simulink model "untitled1"  (R2019b)
(part 13 of 13)

      mask Display: e = 0.06;c1 = [120 150 230]/255;c2 = ([120 150 230]+0)/383;c3 = ([120 150 230]+128)/383;patch([0 1 1 0],[0 0 1 1],c1);patch([0 1 1 1-e 1-e 0+e],[0 0 1 1-e 0+e 0+e],c2);patch([0 0 1 1-e 0+e 0+e],[0 1 1 1-e 1-e 0+e],c3);plot([0 1 1 0 0],[0 0 1 1 0]);disp('weights');
  "IW{2,1}(965,:)'" : Constant  Value=[-0.7144394409110896848602578756981529295444488525390625;0.3471428091304182839138547933544032275676727294921875;0.7770557749069857411683415193692781031131744384765625;0.884710969750206910333645282662473618984222412109375;-0.848870413859076133888947879313491284847259521484375;-0.5348404016948873351822157928836531937122344970703125;0.9006006133464066198968112075817771255970001220703125;0.6799960425277957742906664861948229372501373291015625;-0.4140176799412766950325703874113969504833221435546875;0.9711691691262831493958174178260378539562225341796875]
      mask Display: e = 0.06;c1 = [120 150 230]/255;c2 = ([120 150 230]+0)/383;c3 = ([120 150 230]+128)/383;patch([0 1 1 0],[0 0 1 1],c1);patch([0 1 1 1-e 1-e 0+e],[0 0 1 1-e 0+e 0+e],c2);patch([0 0 1 1-e 0+e 0+e],[0 1 1 1-e 1-e 0+e],c3);plot([0 1 1 0 0],[0 0 1 1 0]);disp('weights');
  "IW{2,1}(966,:)'" : Constant  Value=[-0.01557806455447430238336892216466367244720458984375;-0.5368941087142620194327946592238731682300567626953125;-0.618426386315975573637615525512956082820892333984375;-0.387222706560339080539279166259802877902984619140625;0.6692859941373978660550392305594868957996368408203125;-0.7869100555616228565014580453862436115741729736328125;-0.4994862083211952796801824661088176071643829345703125;-0.5272965717421425058120121320826001465320587158203125;-0.4900147760632862503626938632805831730365753173828125;-0.9665330389173429903593159906449727714061737060546875]
      mask Display: e = 0.06;c1 = [120 150 230]/255;c2 = ([120 150 230]+0)/383;c3 = ([120 150 230]+128)/383;patch([0 1 1 0],[0 0 1 1],c1);patch([0 1 1 1-e 1-e 0+e],[0 0 1 1-e 0+e 0+e],c2);patch([0 0 1 1-e 0+e 0+e],[0 1 1 1-e 1-e 0+e],c3);plot([0 1 1 0 0],[0 0 1 1 0]);disp('weights');
  "IW{2,1}(967,:)'" : Constant  Value=[-0.984051897323352076085711814812384545803070068359375;-0.7181505786073738573094260573270730674266815185546875;0.6028705818402577687464827249641530215740203857421875;-0.3125907138719998812348421779461205005645751953125;-0.646850905156462818723639429663307964801788330078125;-0.1469398150759413379518036890658549964427947998046875;-0.4738723005891622985785716082318685948848724365234375;0.172262093721131659407319602905772626399993896484375;0.1993207325021995046654410543851554393768310546875;-0.698448571765098780161906688590534031391143798828125]
      mask Display: e = 0.06;c1 = [120 150 230]/255;c2 = ([120 150 230]+0)/383;c3 = ([120 150 230]+128)/383;patch([0 1 1 0],[0 0 1 1],c1);patch([0 1 1 1-e 1-e 0+e],[0 0 1 1-e 0+e 0+e],c2);patch([0 0 1 1-e 0+e 0+e],[0 1 1 1-e 1-e 0+e],c3);plot([0 1 1 0 0],[0 0 1 1 0]);disp('weights');
  "IW{2,1}(968,:)'" : Constant  Value=[-0.04533156631802004454812049516476690769195556640625;0.70667647898809438089529066928662359714508056640625;0.1328876134866188163385913867386989295482635498046875;-0.17361026655103017901637940667569637298583984375;-0.040194056538962019686778148752637207508087158203125;-0.256956070446161977116616981220431625843048095703125;0.5707768518799058998780537876882590353488922119140625;0.51234341589951792883539383183233439922332763671875;0.2440885450435192893792191171087324619293212890625;-0.3020562993950519636854323834995739161968231201171875]
      mask Display: e = 0.06;c1 = [120 150 230]/255;c2 = ([120 150 230]+0)/383;c3 = ([120 150 230]+128)/383;patch([0 1 1 0],[0 0 1 1],c1);patch([0 1 1 1-e 1-e 0+e],[0 0 1 1-e 0+e 0+e],c2);patch([0 0 1 1-e 0+e 0+e],[0 1 1 1-e 1-e 0+e],c3);plot([0 1 1 0 0],[0 0 1 1 0]);disp('weights');
  "IW{2,1}(969,:)'" : Constant  Value=[-0.11648547445748480555494097643531858921051025390625;0.4586267717677987576507803169079124927520751953125;-0.511564703530516862173271874780766665935516357421875;-0.1978762319989491036409390289918519556522369384765625;0.324395333392201390410036765388213098049163818359375;0.10679205805803793083441632916219532489776611328125;0.58851580401107117523906708811409771442413330078125;0.24338547710045244087950777611695230007171630859375;0.621085435282426434611124932416714727878570556640625;-0.531323053611133300222491016029380261898040771484375]
      mask Display: e = 0.06;c1 = [120 150 230]/255;c2 = ([120 150 230]+0)/383;c3 = ([120 150 230]+128)/383;patch([0 1 1 0],[0 0 1 1],c1);patch([0 1 1 1-e 1-e 0+e],[0 0 1 1-e 0+e 0+e],c2);patch([0 0 1 1-e 0+e 0+e],[0 1 1 1-e 1-e 0+e],c3);plot([0 1 1 0 0],[0 0 1 1 0]);disp('weights');
  "IW{2,1}(97,:)'" : Constant  Value=[0.5164505764297786516436872261692769825458526611328125;0.98169912664928471457415071199648082256317138671875;-0.0315123656142617392106330953538417816162109375;0.191559320614675510086044596391730010509490966796875;0.996933890817953027863040915690362453460693359375;0.9568910074119532094272244648891501128673553466796875;-0.156110393169701211490973946638405323028564453125;0.5571506750401284957519010276882909238338470458984375;-0.4503567660380503046013700441108085215091705322265625;0.3282242045748076098021783764124847948551177978515625]
      mask Display: e = 0.06;c1 = [120 150 230]/255;c2 = ([120 150 230]+0)/383;c3 = ([120 150 230]+128)/383;patch([0 1 1 0],[0 0 1 1],c1);patch([0 1 1 1-e 1-e 0+e],[0 0 1 1-e 0+e 0+e],c2);patch([0 0 1 1-e 0+e 0+e],[0 1 1 1-e 1-e 0+e],c3);plot([0 1 1 0 0],[0 0 1 1 0]);disp('weights');
  "IW{2,1}(970,:)'" : Constant  Value=[0.66557065240704016417794264270924031734466552734375;-0.342585064829493912696989355026744306087493896484375;-0.330671300947106061585145653225481510162353515625;0.763105148353479645351171711809001863002777099609375;-0.847724061807384909883467116742394864559173583984375;-0.7336611657769716021704198283259756863117218017578125;-0.8233078430220610588463614476495422422885894775390625;0.944306077394880372111174438032321631908416748046875;-0.8467439093702473495994809127296321094036102294921875;0.365460195039065904865083211916498839855194091796875]
      mask Display: e = 0.06;c1 = [120 150 230]/255;c2 = ([120 150 230]+0)/383;c3 = ([120 150 230]+128)/383;patch([0 1 1 0],[0 0 1 1],c1);patch([0 1 1 1-e 1-e 0+e],[0 0 1 1-e 0+e 0+e],c2);patch([0 0 1 1-e 0+e 0+e],[0 1 1 1-e 1-e 0+e],c3);plot([0 1 1 0 0],[0 0 1 1 0]);disp('weights');
  "IW{2,1}(971,:)'" : Constant  Value=[0.09986387496097304250497472821734845638275146484375;-0.83951506989385205059761574375443160533905029296875;0.3955738003209976483276477665640413761138916015625;-0.339458412070430259888098589726723730564117431640625;-0.3938174570716068689790745338541455566883087158203125;-0.5670824324329546417544634095975197851657867431640625;0.1650021316949297212062219841754995286464691162109375;-0.562756802057183147525165622937493026256561279296875;-0.794803053725064767576213853317312896251678466796875;-0.6683564360248277491649560033692978322505950927734375]
      mask Display: e = 0.06;c1 = [120 150 230]/255;c2 = ([120 150 230]+0)/383;c3 = ([120 150 230]+128)/383;patch([0 1 1 0],[0 0 1 1],c1);patch([0 1 1 1-e 1-e 0+e],[0 0 1 1-e 0+e 0+e],c2);patch([0 0 1 1-e 0+e 0+e],[0 1 1 1-e 1-e 0+e],c3);plot([0 1 1 0 0],[0 0 1 1 0]);disp('weights');
  "IW{2,1}(972,:)'" : Constant  Value=[0.268960675494376300065368923242203891277313232421875;0.4899821727860824704947617647121660411357879638671875;0.6479216729186567658160811333800666034221649169921875;0.0558113266099151683619083996745757758617401123046875;-0.6532374748577816081507307899300940334796905517578125;0.8237949914928128780644556172774173319339752197265625;-0.2383918818598125266561282842303626239299774169921875;0.9738616798149990483324245360563509166240692138671875;0.871706348437010003493696785881184041500091552734375;-0.5074443580581782242688859696500003337860107421875]
      mask Display: e = 0.06;c1 = [120 150 230]/255;c2 = ([120 150 230]+0)/383;c3 = ([120 150 230]+128)/383;patch([0 1 1 0],[0 0 1 1],c1);patch([0 1 1 1-e 1-e 0+e],[0 0 1 1-e 0+e 0+e],c2);patch([0 0 1 1-e 0+e 0+e],[0 1 1 1-e 1-e 0+e],c3);plot([0 1 1 0 0],[0 0 1 1 0]);disp('weights');
  "IW{2,1}(973,:)'" : Constant  Value=[0.675627511982876516327678473317064344882965087890625;0.4241577164580718761754951628972776234149932861328125;-0.448557670053332913084886968135833740234375;-0.7164721751960041462581330051762051880359649658203125;-0.2684544674326294622090927077806554734706878662109375;0.54120202347532231357263299287296831607818603515625;0.5901741429993838661260951994336210191249847412109375;-0.2376909062983745268837765252101235091686248779296875;0.285221199923347601412615404115058481693267822265625;0.2521625711384434254114239593036472797393798828125]
      mask Display: e = 0.06;c1 = [120 150 230]/255;c2 = ([120 150 230]+0)/383;c3 = ([120 150 230]+128)/383;patch([0 1 1 0],[0 0 1 1],c1);patch([0 1 1 1-e 1-e 0+e],[0 0 1 1-e 0+e 0+e],c2);patch([0 0 1 1-e 0+e 0+e],[0 1 1 1-e 1-e 0+e],c3);plot([0 1 1 0 0],[0 0 1 1 0]);disp('weights');
  "IW{2,1}(974,:)'" : Constant  Value=[-0.5093344195065017121493156082578934729099273681640625;-0.122100702365118163328361333697102963924407958984375;-0.06613544440721597084120730869472026824951171875;0.85418845517627328689513888093642890453338623046875;0.1864830168329245640990166066330857574939727783203125;-0.1153004956934562397208310358109883964061737060546875;0.7030618126919361277060716020059771835803985595703125;0.9119188834696230205878464403213001787662506103515625;0.0358341940688620130828212495543994009494781494140625;0.2699457411017520680474035543738864362239837646484375]
      mask Display: e = 0.06;c1 = [120 150 230]/255;c2 = ([120 150 230]+0)/383;c3 = ([120 150 230]+128)/383;patch([0 1 1 0],[0 0 1 1],c1);patch([0 1 1 1-e 1-e 0+e],[0 0 1 1-e 0+e 0+e],c2);patch([0 0 1 1-e 0+e 0+e],[0 1 1 1-e 1-e 0+e],c3);plot([0 1 1 0 0],[0 0 1 1 0]);disp('weights');
  "IW{2,1}(975,:)'" : Constant  Value=[-0.44832821462690386482563553727231919765472412109375;-0.581481593458495371606886692461557686328887939453125;-0.8669823002726253502459030642057769000530242919921875;0.4658169283180739750349630412529222667217254638671875;0.9658499535101270350168078948627226054668426513671875;0.554359087851052922957251212210394442081451416015625;0.3636363138170199960086392820812761783599853515625;0.047593285412130370559680159203708171844482421875;0.468161357721236459639158056234009563922882080078125;-0.618507986207100568520900196745060384273529052734375]
      mask Display: e = 0.06;c1 = [120 150 230]/255;c2 = ([120 150 230]+0)/383;c3 = ([120 150 230]+128)/383;patch([0 1 1 0],[0 0 1 1],c1);patch([0 1 1 1-e 1-e 0+e],[0 0 1 1-e 0+e 0+e],c2);patch([0 0 1 1-e 0+e 0+e],[0 1 1 1-e 1-e 0+e],c3);plot([0 1 1 0 0],[0 0 1 1 0]);disp('weights');
  "IW{2,1}(976,:)'" : Constant  Value=[0.63512671701889278352837209240533411502838134765625;0.76995771079419395022114258608780801296234130859375;-0.3323635258169665984695484439725987613201141357421875;0.7269204450465860389840599964372813701629638671875;-0.4794860357969399355937412110506556928157806396484375;0.721878388283787586487960652448236942291259765625;0.5611042141713820097237430672976188361644744873046875;0.5470365148935558696763337138690985739231109619140625;0.524079115559971331350652690161950886249542236328125;0.5223507529721056474869556041085161268711090087890625]
      mask Display: e = 0.06;c1 = [120 150 230]/255;c2 = ([120 150 230]+0)/383;c3 = ([120 150 230]+128)/383;patch([0 1 1 0],[0 0 1 1],c1);patch([0 1 1 1-e 1-e 0+e],[0 0 1 1-e 0+e 0+e],c2);patch([0 0 1 1-e 0+e 0+e],[0 1 1 1-e 1-e 0+e],c3);plot([0 1 1 0 0],[0 0 1 1 0]);disp('weights');
  "IW{2,1}(977,:)'" : Constant  Value=[-0.661425562563644486857583615346811711788177490234375;0.881450618622593662365716227213852107524871826171875;0.5362793846547531106949691093177534639835357666015625;0.9636728247019397119998984635458327829837799072265625;-0.6788919886295976535706131471670232713222503662109375;-0.2454345244011097992853365212795324623584747314453125;-0.2134483663315069890131780994124710559844970703125;-0.507588810722410244125057943165302276611328125;-0.0191293381497643633082361702690832316875457763671875;0.1988419730259847195696920607588253915309906005859375]
      mask Display: e = 0.06;c1 = [120 150 230]/255;c2 = ([120 150 230]+0)/383;c3 = ([120 150 230]+128)/383;patch([0 1 1 0],[0 0 1 1],c1);patch([0 1 1 1-e 1-e 0+e],[0 0 1 1-e 0+e 0+e],c2);patch([0 0 1 1-e 0+e 0+e],[0 1 1 1-e 1-e 0+e],c3);plot([0 1 1 0 0],[0 0 1 1 0]);disp('weights');
  "IW{2,1}(978,:)'" : Constant  Value=[0.9397617197588667981023036190890707075595855712890625;-0.5050778654996699312818009275360964238643646240234375;-0.2310095659395277056802342485752888023853302001953125;-0.72151071109553921445467494777403771877288818359375;0.2458828822041303485690377783612348139286041259765625;-0.6318146365362140581822814056067727506160736083984375;0.493954060451254672869936257484368979930877685546875;-0.039417507091375370009700418449938297271728515625;-0.9730967142666300251363509232760407030582427978515625;-0.8911115925057833120348504962748847901821136474609375]
      mask Display: e = 0.06;c1 = [120 150 230]/255;c2 = ([120 150 230]+0)/383;c3 = ([120 150 230]+128)/383;patch([0 1 1 0],[0 0 1 1],c1);patch([0 1 1 1-e 1-e 0+e],[0 0 1 1-e 0+e 0+e],c2);patch([0 0 1 1-e 0+e 0+e],[0 1 1 1-e 1-e 0+e],c3);plot([0 1 1 0 0],[0 0 1 1 0]);disp('weights');
  "IW{2,1}(979,:)'" : Constant  Value=[-0.4741075419004106006326537681161426007747650146484375;0.205108870171887058830861860769800841808319091796875;0.29256486552897253972105318098329007625579833984375;0.7587563553566012419793196386308409273624420166015625;-0.375454775245055660803927821689285337924957275390625;0.231516223087936179325652119587175548076629638671875;0.070654245879933075258350072544999420642852783203125;0.83413919498149358133787245606072247028350830078125;0.6313603211407159410128997478750534355640411376953125;-0.85603804792848148252915052580647170543670654296875]
      mask Display: e = 0.06;c1 = [120 150 230]/255;c2 = ([120 150 230]+0)/383;c3 = ([120 150 230]+128)/383;patch([0 1 1 0],[0 0 1 1],c1);patch([0 1 1 1-e 1-e 0+e],[0 0 1 1-e 0+e 0+e],c2);patch([0 0 1 1-e 0+e 0+e],[0 1 1 1-e 1-e 0+e],c3);plot([0 1 1 0 0],[0 0 1 1 0]);disp('weights');
  "IW{2,1}(98,:)'" : Constant  Value=[-0.7749528854198344252068864079774357378482818603515625;-0.7248848268697927199610830939491279423236846923828125;-0.9015271498971679786649247034802101552486419677734375;0.3448050374539517459737680837861262261867523193359375;0.86952403079192475132686013239435851573944091796875;0.767582231090413902308000615448690950870513916015625;-0.64782980375393339755873967078514397144317626953125;0.517582748277408466464066805201582610607147216796875;0.9891107209328253713209733177791349589824676513671875;0.391932819643511454188455900293774902820587158203125]
      mask Display: e = 0.06;c1 = [120 150 230]/255;c2 = ([120 150 230]+0)/383;c3 = ([120 150 230]+128)/383;patch([0 1 1 0],[0 0 1 1],c1);patch([0 1 1 1-e 1-e 0+e],[0 0 1 1-e 0+e 0+e],c2);patch([0 0 1 1-e 0+e 0+e],[0 1 1 1-e 1-e 0+e],c3);plot([0 1 1 0 0],[0 0 1 1 0]);disp('weights');
  "IW{2,1}(980,:)'" : Constant  Value=[-0.79147398202981111836606942233629524707794189453125;0.2718975678685253694055745654623024165630340576171875;-0.4094504931238824863015679511590860784053802490234375;0.81854986253682682217913679778575897216796875;0.605274059499623096058940063812769949436187744140625;0.63404117958328409798696156940422952175140380859375;0.6294911340532147736581691788160242140293121337890625;-0.1480106713086433156689736279076896607875823974609375;0.93064947410425968854497114080004394054412841796875;0.93956211150475343885091206175275146961212158203125]
      mask Display: e = 0.06;c1 = [120 150 230]/255;c2 = ([120 150 230]+0)/383;c3 = ([120 150 230]+128)/383;patch([0 1 1 0],[0 0 1 1],c1);patch([0 1 1 1-e 1-e 0+e],[0 0 1 1-e 0+e 0+e],c2);patch([0 0 1 1-e 0+e 0+e],[0 1 1 1-e 1-e 0+e],c3);plot([0 1 1 0 0],[0 0 1 1 0]);disp('weights');
  "IW{2,1}(981,:)'" : Constant  Value=[-0.0852692222631059593140889774076640605926513671875;-0.899091542873903026844573105336166918277740478515625;-0.1471286623457948028459441047743894159793853759765625;-0.4211931943745510498189332793117500841617584228515625;0.36330329234651781433740325155667960643768310546875;-0.139104176957447922546862173476256430149078369140625;-0.7284662842966298512692446820437908172607421875;0.873058432394929528896909687318839132785797119140625;-0.605449246597180579243513420806266367435455322265625;-0.3582669903376476394640803846414200961589813232421875]
      mask Display: e = 0.06;c1 = [120 150 230]/255;c2 = ([120 150 230]+0)/383;c3 = ([120 150 230]+128)/383;patch([0 1 1 0],[0 0 1 1],c1);patch([0 1 1 1-e 1-e 0+e],[0 0 1 1-e 0+e 0+e],c2);patch([0 0 1 1-e 0+e 0+e],[0 1 1 1-e 1-e 0+e],c3);plot([0 1 1 0 0],[0 0 1 1 0]);disp('weights');
  "IW{2,1}(982,:)'" : Constant  Value=[-0.4342255528810079479029582216753624379634857177734375;0.172996624453667369181175672565586864948272705078125;0.2102942438550774451044844681746326386928558349609375;0.125405454503676683231105926097370684146881103515625;-0.9632340007484112565094847013824619352817535400390625;0.01979000329602786933946845238097012042999267578125;0.718517973057300363137755994102917611598968505859375;-0.358865564478632936840085676521994173526763916015625;0.3435920013824065311069944073096849024295806884765625;0.17049996845140835688425795524381101131439208984375]
      mask Display: e = 0.06;c1 = [120 150 230]/255;c2 = ([120 150 230]+0)/383;c3 = ([120 150 230]+128)/383;patch([0 1 1 0],[0 0 1 1],c1);patch([0 1 1 1-e 1-e 0+e],[0 0 1 1-e 0+e 0+e],c2);patch([0 0 1 1-e 0+e 0+e],[0 1 1 1-e 1-e 0+e],c3);plot([0 1 1 0 0],[0 0 1 1 0]);disp('weights');
  "IW{2,1}(983,:)'" : Constant  Value=[-0.1677270431949711149144377486663870513439178466796875;0.181662621682935565559091628529131412506103515625;0.851057986800337840094243802013806998729705810546875;-0.072748429997369523647421374334953725337982177734375;0.7882143648824444515099685304448939859867095947265625;0.4502981756526995837930371635593473911285400390625;0.1336104762519625399619371819426305592060089111328125;-0.9894179168451724404320657413336448371410369873046875;-0.60904986299242214187188437790609896183013916015625;0.555950035385905483309443297912366688251495361328125]
      mask Display: e = 0.06;c1 = [120 150 230]/255;c2 = ([120 150 230]+0)/383;c3 = ([120 150 230]+128)/383;patch([0 1 1 0],[0 0 1 1],c1);patch([0 1 1 1-e 1-e 0+e],[0 0 1 1-e 0+e 0+e],c2);patch([0 0 1 1-e 0+e 0+e],[0 1 1 1-e 1-e 0+e],c3);plot([0 1 1 0 0],[0 0 1 1 0]);disp('weights');
  "IW{2,1}(984,:)'" : Constant  Value=[-0.9698249573309529747433543889201246201992034912109375;-0.234376616891645017659584482316859066486358642578125;0.9737840786331359854699485367746092379093170166015625;0.8760765465004822782901783284614793956279754638671875;-0.024687881459021010499554904527030885219573974609375;-0.7129955988575460423817276023328304290771484375;-0.834665311211235660948659642599523067474365234375;0.838502337609266401585728090140037238597869873046875;0.8558601766537587973715517364325933158397674560546875;0.6368968800970955523865768554969690740108489990234375]
      mask Display: e = 0.06;c1 = [120 150 230]/255;c2 = ([120 150 230]+0)/383;c3 = ([120 150 230]+128)/383;patch([0 1 1 0],[0 0 1 1],c1);patch([0 1 1 1-e 1-e 0+e],[0 0 1 1-e 0+e 0+e],c2);patch([0 0 1 1-e 0+e 0+e],[0 1 1 1-e 1-e 0+e],c3);plot([0 1 1 0 0],[0 0 1 1 0]);disp('weights');
  "IW{2,1}(985,:)'" : Constant  Value=[-0.0091677671380521186250689424923621118068695068359375;0.800228653495768327275072806514799594879150390625;0.5410823945520999433966835567844100296497344970703125;-0.9494611157890806563131036455160938203334808349609375;-0.659980658289798238769208182930015027523040771484375;-0.00114901150523305517481276183389127254486083984375;-0.0136490491228522525801736264838837087154388427734375;-0.319972954472963255767581358668394386768341064453125;0.83703066722275121236407358082942664623260498046875;-0.444610457951165383150282650603912770748138427734375]
      mask Display: e = 0.06;c1 = [120 150 230]/255;c2 = ([120 150 230]+0)/383;c3 = ([120 150 230]+128)/383;patch([0 1 1 0],[0 0 1 1],c1);patch([0 1 1 1-e 1-e 0+e],[0 0 1 1-e 0+e 0+e],c2);patch([0 0 1 1-e 0+e 0+e],[0 1 1 1-e 1-e 0+e],c3);plot([0 1 1 0 0],[0 0 1 1 0]);disp('weights');
  "IW{2,1}(986,:)'" : Constant  Value=[0.8297443864155129578108471832820214331150054931640625;0.363935670188301418903620287892408668994903564453125;0.100383258658132579199673273251391947269439697265625;0.68812431176497401708047618740238249301910400390625;0.39841482140100747955102633568458259105682373046875;-0.5389940279242357856759326750761829316616058349609375;0.942748456213683194704344714409671723842620849609375;0.9881289869271363546232578300987370312213897705078125;-0.40606747251954455890654571703635156154632568359375;0.4138975726274001232241062098182737827301025390625]
      mask Display: e = 0.06;c1 = [120 150 230]/255;c2 = ([120 150 230]+0)/383;c3 = ([120 150 230]+128)/383;patch([0 1 1 0],[0 0 1 1],c1);patch([0 1 1 1-e 1-e 0+e],[0 0 1 1-e 0+e 0+e],c2);patch([0 0 1 1-e 0+e 0+e],[0 1 1 1-e 1-e 0+e],c3);plot([0 1 1 0 0],[0 0 1 1 0]);disp('weights');
  "IW{2,1}(987,:)'" : Constant  Value=[-0.99506550776042868022841503261588513851165771484375;0.68389640586497879581884262734092772006988525390625;-0.2268259999791315539852121219155378639698028564453125;-0.957738642747987256598207750357687473297119140625;0.26389345282455511920716162421740591526031494140625;-0.6102323831253475550084885981050319969654083251953125;-0.927066660789935159669994391151703894138336181640625;-0.549182384059821782074095608550123870372772216796875;0.0328332951849941157007606307161040604114532470703125;0.095697283614887940217386130825616419315338134765625]
      mask Display: e = 0.06;c1 = [120 150 230]/255;c2 = ([120 150 230]+0)/383;c3 = ([120 150 230]+128)/383;patch([0 1 1 0],[0 0 1 1],c1);patch([0 1 1 1-e 1-e 0+e],[0 0 1 1-e 0+e 0+e],c2);patch([0 0 1 1-e 0+e 0+e],[0 1 1 1-e 1-e 0+e],c3);plot([0 1 1 0 0],[0 0 1 1 0]);disp('weights');
  "IW{2,1}(988,:)'" : Constant  Value=[0.69592152169732468536267333547584712505340576171875;0.741406290005517387697864251094870269298553466796875;-0.8585444882144399603163265055627562105655670166015625;0.00846499148783852461974674952216446399688720703125;0.7336265843222864457828791273641400039196014404296875;-0.14664201888037897703043199726380407810211181640625;0.679580078540876542092519230209290981292724609375;-0.4031972201373006381430741384974680840969085693359375;-0.7367485188008242591450880354386754333972930908203125;-0.6177617192172204507727428790531121194362640380859375]
      mask Display: e = 0.06;c1 = [120 150 230]/255;c2 = ([120 150 230]+0)/383;c3 = ([120 150 230]+128)/383;patch([0 1 1 0],[0 0 1 1],c1);patch([0 1 1 1-e 1-e 0+e],[0 0 1 1-e 0+e 0+e],c2);patch([0 0 1 1-e 0+e 0+e],[0 1 1 1-e 1-e 0+e],c3);plot([0 1 1 0 0],[0 0 1 1 0]);disp('weights');
  "IW{2,1}(989,:)'" : Constant  Value=[0.5258405630769544814029359258711338043212890625;0.02362857811346774639105206006206572055816650390625;0.591850556674113903454781393520534038543701171875;-0.6811184003189232338826286650146357715129852294921875;0.8849967885033940273586949842865578830242156982421875;-0.1936775865755897552134001671220175921916961669921875;0.583123188590920715768106674659065902233123779296875;0.656936314591705095011775483726523816585540771484375;-0.7871214385727558493499600444920361042022705078125;-0.575571636359800908877559777465648949146270751953125]
      mask Display: e = 0.06;c1 = [120 150 230]/255;c2 = ([120 150 230]+0)/383;c3 = ([120 150 230]+128)/383;patch([0 1 1 0],[0 0 1 1],c1);patch([0 1 1 1-e 1-e 0+e],[0 0 1 1-e 0+e 0+e],c2);patch([0 0 1 1-e 0+e 0+e],[0 1 1 1-e 1-e 0+e],c3);plot([0 1 1 0 0],[0 0 1 1 0]);disp('weights');
  "IW{2,1}(99,:)'" : Constant  Value=[0.575150520088075101199365235515870153903961181640625;0.37465909921554629846696116146631538867950439453125;-0.218631460734588500827157986350357532501220703125;0.7537750788373838162215179181657731533050537109375;0.018582050865799448757798018050380051136016845703125;0.7600810117561043188771918721613474190235137939453125;-0.76860054930705512532540524262003600597381591796875;-0.94039249795119328467762898071669042110443115234375;-0.3834774356905821246499499466153793036937713623046875;-0.3101774619584951597772715103928931057453155517578125]
      mask Display: e = 0.06;c1 = [120 150 230]/255;c2 = ([120 150 230]+0)/383;c3 = ([120 150 230]+128)/383;patch([0 1 1 0],[0 0 1 1],c1);patch([0 1 1 1-e 1-e 0+e],[0 0 1 1-e 0+e 0+e],c2);patch([0 0 1 1-e 0+e 0+e],[0 1 1 1-e 1-e 0+e],c3);plot([0 1 1 0 0],[0 0 1 1 0]);disp('weights');
  "IW{2,1}(990,:)'" : Constant  Value=[0.2326555017398941327400052614393644034862518310546875;-0.816916889396598566719376321998424828052520751953125;-0.9732908311802408451995916038868017494678497314453125;-0.3538488035342648441172741513582877814769744873046875;-0.653900547497509254668557332479394972324371337890625;0.4942587994270748463776499193045310676097869873046875;-0.337155697405948640010819872259162366390228271484375;0.9385189605570951609792018643929623067378997802734375;0.13364804997201940039985856856219470500946044921875;-0.61969961094390324518599300063215196132659912109375]
      mask Display: e = 0.06;c1 = [120 150 230]/255;c2 = ([120 150 230]+0)/383;c3 = ([120 150 230]+128)/383;patch([0 1 1 0],[0 0 1 1],c1);patch([0 1 1 1-e 1-e 0+e],[0 0 1 1-e 0+e 0+e],c2);patch([0 0 1 1-e 0+e 0+e],[0 1 1 1-e 1-e 0+e],c3);plot([0 1 1 0 0],[0 0 1 1 0]);disp('weights');
  "IW{2,1}(991,:)'" : Constant  Value=[-0.9871028878722487576169442036189138889312744140625;0.5265970638336383569111376345972530543804168701171875;-0.0364342149465277653774819555110298097133636474609375;-0.1658721641537710400626792761613614857196807861328125;-0.28175363874287295828935384633950889110565185546875;0.1596594056545324047391432031872682273387908935546875;0.5156289048657594076274790495517663657665252685546875;-0.04013802190475512787770639988593757152557373046875;0.26539842067519447965651124832220375537872314453125;-0.1596961057493351265890169088379479944705963134765625]
      mask Display: e = 0.06;c1 = [120 150 230]/255;c2 = ([120 150 230]+0)/383;c3 = ([120 150 230]+128)/383;patch([0 1 1 0],[0 0 1 1],c1);patch([0 1 1 1-e 1-e 0+e],[0 0 1 1-e 0+e 0+e],c2);patch([0 0 1 1-e 0+e 0+e],[0 1 1 1-e 1-e 0+e],c3);plot([0 1 1 0 0],[0 0 1 1 0]);disp('weights');
  "IW{2,1}(992,:)'" : Constant  Value=[-0.938491924689132783754530464648269116878509521484375;0.13752241605833770421440931386314332485198974609375;-0.879241846972659946146677611977793276309967041015625;0.660907937722420069093232086743228137493133544921875;-0.8805833917143324196530329572851769626140594482421875;0.8707162146279545655858100872137583792209625244140625;0.7183941091036754045262568979524075984954833984375;0.7690132988575839600997596789966337382793426513671875;-0.6880816901412176722629965297528542578220367431640625;-0.17645370421463635324244023649953305721282958984375]
      mask Display: e = 0.06;c1 = [120 150 230]/255;c2 = ([120 150 230]+0)/383;c3 = ([120 150 230]+128)/383;patch([0 1 1 0],[0 0 1 1],c1);patch([0 1 1 1-e 1-e 0+e],[0 0 1 1-e 0+e 0+e],c2);patch([0 0 1 1-e 0+e 0+e],[0 1 1 1-e 1-e 0+e],c3);plot([0 1 1 0 0],[0 0 1 1 0]);disp('weights');
  "IW{2,1}(993,:)'" : Constant  Value=[-0.4980607181836622654458324177539907395839691162109375;0.0352171225070898596953838932677172124385833740234375;-0.9022465883082320114993990500806830823421478271484375;0.6565955652422099664278221098356880247592926025390625;-0.0859885417955921216304204790503717958927154541015625;-0.387275276261659140430992920300923287868499755859375;0.17376291985281344665281721972860395908355712890625;-0.633859314112658278617118412512354552745819091796875;-0.912910598277362428376591196865774691104888916015625;-0.371211006578622715323945158161222934722900390625]
      mask Display: e = 0.06;c1 = [120 150 230]/255;c2 = ([120 150 230]+0)/383;c3 = ([120 150 230]+128)/383;patch([0 1 1 0],[0 0 1 1],c1);patch([0 1 1 1-e 1-e 0+e],[0 0 1 1-e 0+e 0+e],c2);patch([0 0 1 1-e 0+e 0+e],[0 1 1 1-e 1-e 0+e],c3);plot([0 1 1 0 0],[0 0 1 1 0]);disp('weights');
  "IW{2,1}(994,:)'" : Constant  Value=[0.716418706487937928528708653175272047519683837890625;0.9078608278320932090110773060587234795093536376953125;-0.2241622493210202460289792725234292447566986083984375;-0.615222801058393553574887846480123698711395263671875;-0.8160012056376551026204424488241784274578094482421875;0.370799994036933089347485292819328606128692626953125;0.2508144711549114003190652510966174304485321044921875;0.736621451000748717063970616436563432216644287109375;0.806232100812742213946648917044512927532196044921875;-0.156100428614929231940777754061855375766754150390625]
      mask Display: e = 0.06;c1 = [120 150 230]/255;c2 = ([120 150 230]+0)/383;c3 = ([120 150 230]+128)/383;patch([0 1 1 0],[0 0 1 1],c1);patch([0 1 1 1-e 1-e 0+e],[0 0 1 1-e 0+e 0+e],c2);patch([0 0 1 1-e 0+e 0+e],[0 1 1 1-e 1-e 0+e],c3);plot([0 1 1 0 0],[0 0 1 1 0]);disp('weights');
  "IW{2,1}(995,:)'" : Constant  Value=[-0.1364054153193647866970650284201838076114654541015625;0.4749016071199445576667130808345973491668701171875;0.0627837665431270064431146238348446786403656005859375;-0.94389294827828518208434616099111735820770263671875;0.5376715319352303179556429313379339873790740966796875;-0.0367819040713797118513639361481182277202606201171875;-0.6680869617124221004900164189166389405727386474609375;-0.4980836665759216241866624841350130736827850341796875;-0.53400854447419821013909313478507101535797119140625;0.541155799376516366550049497163854539394378662109375]
      mask Display: e = 0.06;c1 = [120 150 230]/255;c2 = ([120 150 230]+0)/383;c3 = ([120 150 230]+128)/383;patch([0 1 1 0],[0 0 1 1],c1);patch([0 1 1 1-e 1-e 0+e],[0 0 1 1-e 0+e 0+e],c2);patch([0 0 1 1-e 0+e 0+e],[0 1 1 1-e 1-e 0+e],c3);plot([0 1 1 0 0],[0 0 1 1 0]);disp('weights');
  "IW{2,1}(996,:)'" : Constant  Value=[0.5430783261647318393983141504577361047267913818359375;-0.170378059408950566222529232618398964405059814453125;0.6296517543088218094027297411230392754077911376953125;-0.918593485775859530662046381621621549129486083984375;-0.9230395235992363556221107501187361776828765869140625;0.36388216711752630061482705059461295604705810546875;0.1324210930120364171358460225746966898441314697265625;-0.0746117057159789709430697257630527019500732421875;-0.0607336809067546834484119244734756648540496826171875;0.656421764498073212479312132927589118480682373046875]
      mask Display: e = 0.06;c1 = [120 150 230]/255;c2 = ([120 150 230]+0)/383;c3 = ([120 150 230]+128)/383;patch([0 1 1 0],[0 0 1 1],c1);patch([0 1 1 1-e 1-e 0+e],[0 0 1 1-e 0+e 0+e],c2);patch([0 0 1 1-e 0+e 0+e],[0 1 1 1-e 1-e 0+e],c3);plot([0 1 1 0 0],[0 0 1 1 0]);disp('weights');
  "IW{2,1}(997,:)'" : Constant  Value=[-0.26686842394291421243224249337799847126007080078125;0.8418202530941545358444955127197317779064178466796875;0.9659680681210700559091719696880318224430084228515625;-0.3622829569550585215864657584461383521556854248046875;-0.5596994386348514982643109760829247534275054931640625;-0.4700339909179993558296928313211537897586822509765625;-0.735542729375474824138336771284230053424835205078125;0.630837394791175398722771205939352512359619140625;-0.1048472410461276371762551207211799919605255126953125;-0.2478265302792355129213319742120802402496337890625]
      mask Display: e = 0.06;c1 = [120 150 230]/255;c2 = ([120 150 230]+0)/383;c3 = ([120 150 230]+128)/383;patch([0 1 1 0],[0 0 1 1],c1);patch([0 1 1 1-e 1-e 0+e],[0 0 1 1-e 0+e 0+e],c2);patch([0 0 1 1-e 0+e 0+e],[0 1 1 1-e 1-e 0+e],c3);plot([0 1 1 0 0],[0 0 1 1 0]);disp('weights');
  "IW{2,1}(998,:)'" : Constant  Value=[0.4166831148598288958595503572723828256130218505859375;0.2389745795749067536206666773068718612194061279296875;0.530581258375642850211306722485460340976715087890625;-0.2475053544910454927929777113604359328746795654296875;-0.1220999443843162612921560139511711895465850830078125;0.1101426816156390042777957205544225871562957763671875;0.736631290047672138143752817995846271514892578125;0.3962806090034616257611332912347279489040374755859375;0.977449407102380263268059934489428997039794921875;-0.72303125884767904807404192979447543621063232421875]
      mask Display: e = 0.06;c1 = [120 150 230]/255;c2 = ([120 150 230]+0)/383;c3 = ([120 150 230]+128)/383;patch([0 1 1 0],[0 0 1 1],c1);patch([0 1 1 1-e 1-e 0+e],[0 0 1 1-e 0+e 0+e],c2);patch([0 0 1 1-e 0+e 0+e],[0 1 1 1-e 1-e 0+e],c3);plot([0 1 1 0 0],[0 0 1 1 0]);disp('weights');
  "IW{2,1}(999,:)'" : Constant  Value=[-0.533189763526342286326098474091850221157073974609375;0.109347486515975589327354100532829761505126953125;-0.09315402580937615084621938876807689666748046875;0.6066138928676629848979473536019213497638702392578125;-0.700926596028907500368632099707610905170440673828125;0.1784918690411496644543376532965339720249176025390625;-0.44436022505788042025187678518705070018768310546875;-0.128909807311281543462655463372357189655303955078125;-0.5423537750827656100938156669144518673419952392578125;-0.950914322250334453912046228651888668537139892578125]
      mask Display: e = 0.06;c1 = [120 150 230]/255;c2 = ([120 150 230]+0)/383;c3 = ([120 150 230]+128)/383;patch([0 1 1 0],[0 0 1 1],c1);patch([0 1 1 1-e 1-e 0+e],[0 0 1 1-e 0+e 0+e],c2);patch([0 0 1 1-e 0+e 0+e],[0 1 1 1-e 1-e 0+e],c3);plot([0 1 1 0 0],[0 0 1 1 0]);disp('weights');
  Mux : Mux  Inputs=1001
      mask Display: e = 0.06;c1 = [120 150 230]/255;c2 = ([120 150 230]+0)/383;c3 = ([120 150 230]+128)/383;patch([0 1 1 0],[0 0 1 1],c1);patch([0 1 1 1-e 1-e 0+e],[0 0 1 1-e 0+e 0+e],c2);patch([0 0 1 1-e 0+e 0+e],[0 1 1 1-e 1-e 0+e],c3);plot([0 1 1 0 0],[0 0 1 1 0]);disp('Mux');
  dotprod{1..1001} (1001 alike) : neural/Weight Functions/dotprod
      settings: SourceProductName=Deep Learning Toolbox
  "lz{2,1}" : Outport
      mask Display: e = 0.06;c1 = [120 230 180]/255;c2 = ([120 230 180]+0)/(256+128);c3 = ([120 230 180]+128)/(256+128);patch([0 1 1 0],[0 0 1 1],c1);patch([0 1 1 1-e 1-e 0+e],[0 0 1 1-e 0+e 0+e],c2);patch([0 0 1 1-e 0+e 0+e],[0 1 1 1-e 1-e 0+e],c3);plot([0 1 1 0 0],[0 0 1 1 0]);
  wires:
  "IW{2,1}(1,:)'"/1 -> dotprod1/1
  "ad{2,1}"/1 -> dotprod1/2, dotprod2/2, dotprod3/2, dotprod4/2, dotprod5/2, dotprod6/2, dotprod7/2, dotprod8/2, dotprod9/2, dotprod10/2, dotprod11/2, dotprod12/2, dotprod13/2, dotprod14/2, dotprod15/2, dotprod16/2, dotprod17/2, dotprod18/2, dotprod19/2, dotprod20/2, dotprod21/2, dotprod22/2, dotprod23/2, dotprod24/2, dotprod25/2, dotprod26/2, dotprod27/2, dotprod28/2, dotprod29/2, dotprod30/2, dotprod31/2, dotprod32/2, dotprod33/2, dotprod34/2, dotprod35/2, dotprod36/2, dotprod37/2, dotprod38/2, dotprod39/2, dotprod40/2, dotprod41/2, dotprod42/2, dotprod43/2, dotprod44/2, dotprod45/2, dotprod46/2, dotprod47/2, dotprod48/2, dotprod49/2, dotprod50/2, dotprod51/2, dotprod52/2, dotprod53/2, dotprod54/2, dotprod55/2, dotprod56/2, dotprod57/2, dotprod58/2, dotprod59/2, dotprod60/2, dotprod61/2, dotprod62/2, dotprod63/2, dotprod64/2, dotprod65/2, dotprod66/2, dotprod67/2, dotprod68/2, dotprod69/2, dotprod70/2, dotprod71/2, dotprod72/2, dotprod73/2, dotprod74/2, dotprod75/2, dotprod76/2, dotprod77/2, dotprod78/2, dotprod79/2, dotprod80/2, dotprod81/2, dotprod82/2, dotprod83/2, dotprod84/2, dotprod85/2, dotprod86/2, dotprod87/2, dotprod88/2, dotprod89/2, dotprod90/2, dotprod91/2, dotprod92/2, dotprod93/2, dotprod94/2, dotprod95/2, dotprod96/2, dotprod97/2, dotprod98/2, dotprod99/2, dotprod100/2, dotprod101/2, dotprod102/2, dotprod103/2, dotprod104/2, dotprod105/2, dotprod106/2, dotprod107/2, dotprod108/2, dotprod109/2, dotprod110/2, dotprod111/2, dotprod112/2, dotprod113/2, dotprod114/2, dotprod115/2, dotprod116/2, dotprod117/2, dotprod118/2, dotprod119/2, dotprod120/2, dotprod121/2, dotprod122/2, dotprod123/2, dotprod124/2, dotprod125/2, dotprod126/2, dotprod127/2, dotprod128/2, dotprod129/2, dotprod130/2, dotprod131/2, dotprod132/2, dotprod133/2, dotprod134/2, dotprod135/2, dotprod136/2, dotprod137/2, dotprod138/2, dotprod139/2, dotprod140/2, dotprod141/2, dotprod142/2, dotprod143/2, dotprod144/2, dotprod145/2, dotprod146/2, dotprod147/2, dotprod148/2, dotprod149/2, dotprod150/2, dotprod151/2, dotprod152/2, dotprod153/2, dotprod154/2, dotprod155/2, dotprod156/2, dotprod157/2, dotprod158/2, dotprod159/2, dotprod160/2, dotprod161/2, dotprod162/2, dotprod163/2, dotprod164/2, dotprod165/2, dotprod166/2, dotprod167/2, dotprod168/2, dotprod169/2, dotprod170/2, dotprod171/2, dotprod172/2, dotprod173/2, dotprod174/2, dotprod175/2, dotprod176/2, dotprod177/2, dotprod178/2, dotprod179/2, dotprod180/2, dotprod181/2, dotprod182/2, dotprod183/2, dotprod184/2, dotprod185/2, dotprod186/2, dotprod187/2, dotprod188/2, dotprod189/2, dotprod190/2, dotprod191/2, dotprod192/2, dotprod193/2, dotprod194/2, dotprod195/2, dotprod196/2, dotprod197/2, dotprod198/2, dotprod199/2, dotprod200/2, dotprod201/2, dotprod202/2, dotprod203/2, dotprod204/2, dotprod205/2, dotprod206/2, dotprod207/2, dotprod208/2, dotprod209/2, dotprod210/2, dotprod211/2, dotprod212/2, dotprod213/2, dotprod214/2, dotprod215/2, dotprod216/2, dotprod217/2, dotprod218/2, dotprod219/2, dotprod220/2, dotprod221/2, dotprod222/2, dotprod223/2, dotprod224/2, dotprod225/2, dotprod226/2, dotprod227/2, dotprod228/2, dotprod229/2, dotprod230/2, dotprod231/2, dotprod232/2, dotprod233/2, dotprod234/2, dotprod235/2, dotprod236/2, dotprod237/2, dotprod238/2, dotprod239/2, dotprod240/2, dotprod241/2, dotprod242/2, dotprod243/2, dotprod244/2, dotprod245/2, dotprod246/2, dotprod247/2, dotprod248/2, dotprod249/2, dotprod250/2, dotprod251/2, dotprod252/2, dotprod253/2, dotprod254/2, dotprod255/2, dotprod256/2, dotprod257/2, dotprod258/2, dotprod259/2, dotprod260/2, dotprod261/2, dotprod262/2, dotprod263/2, dotprod264/2, dotprod265/2, dotprod266/2, dotprod267/2, dotprod268/2, dotprod269/2, dotprod270/2, dotprod271/2, dotprod272/2, dotprod273/2, dotprod274/2, dotprod275/2, dotprod276/2, dotprod277/2, dotprod278/2, dotprod279/2, dotprod280/2, dotprod281/2, dotprod282/2, dotprod283/2, dotprod284/2, dotprod285/2, dotprod286/2, dotprod287/2, dotprod288/2, dotprod289/2, dotprod290/2, dotprod291/2, dotprod292/2, dotprod293/2, dotprod294/2, dotprod295/2, dotprod296/2, dotprod297/2, dotprod298/2, dotprod299/2, dotprod300/2, dotprod301/2, dotprod302/2, dotprod303/2, dotprod304/2, dotprod305/2, dotprod306/2, dotprod307/2, dotprod308/2, dotprod309/2, dotprod310/2, dotprod311/2, dotprod312/2, dotprod313/2, dotprod314/2, dotprod315/2, dotprod316/2, dotprod317/2, dotprod318/2, dotprod319/2, dotprod320/2, dotprod321/2, dotprod322/2, dotprod323/2, dotprod324/2, dotprod325/2, dotprod326/2, dotprod327/2, dotprod328/2, dotprod329/2, dotprod330/2, dotprod331/2, dotprod332/2, dotprod333/2, dotprod334/2, dotprod335/2, dotprod336/2, dotprod337/2, dotprod338/2, dotprod339/2, dotprod340/2, dotprod341/2, dotprod342/2, dotprod343/2, dotprod344/2, dotprod345/2, dotprod346/2, dotprod347/2, dotprod348/2, dotprod349/2, dotprod350/2, dotprod351/2, dotprod352/2, dotprod353/2, dotprod354/2, dotprod355/2, dotprod356/2, dotprod357/2, dotprod358/2, dotprod359/2, dotprod360/2, dotprod361/2, dotprod362/2, dotprod363/2, dotprod364/2, dotprod365/2, dotprod366/2, dotprod367/2, dotprod368/2, dotprod369/2, dotprod370/2, dotprod371/2, dotprod372/2, dotprod373/2, dotprod374/2, dotprod375/2, dotprod376/2, dotprod377/2, dotprod378/2, dotprod379/2, dotprod380/2, dotprod381/2, dotprod382/2, dotprod383/2, dotprod384/2, dotprod385/2, dotprod386/2, dotprod387/2, dotprod388/2, dotprod389/2, dotprod390/2, dotprod391/2, dotprod392/2, dotprod393/2, dotprod394/2, dotprod395/2, dotprod396/2, dotprod397/2, dotprod398/2, dotprod399/2, dotprod400/2, dotprod401/2, dotprod402/2, dotprod403/2, dotprod404/2, dotprod405/2, dotprod406/2, dotprod407/2, dotprod408/2, dotprod409/2, dotprod410/2, dotprod411/2, dotprod412/2, dotprod413/2, dotprod414/2, dotprod415/2, dotprod416/2, dotprod417/2, dotprod418/2, dotprod419/2, dotprod420/2, dotprod421/2, dotprod422/2, dotprod423/2, dotprod424/2, dotprod425/2, dotprod426/2, dotprod427/2, dotprod428/2, dotprod429/2, dotprod430/2, dotprod431/2, dotprod432/2, dotprod433/2, dotprod434/2, dotprod435/2, dotprod436/2, dotprod437/2, dotprod438/2, dotprod439/2, dotprod440/2, dotprod441/2, dotprod442/2, dotprod443/2, dotprod444/2, dotprod445/2, dotprod446/2, dotprod447/2, dotprod448/2, dotprod449/2, dotprod450/2, dotprod451/2, dotprod452/2, dotprod453/2, dotprod454/2, dotprod455/2, dotprod456/2, dotprod457/2, dotprod458/2, dotprod459/2, dotprod460/2, dotprod461/2, dotprod462/2, dotprod463/2, dotprod464/2, dotprod465/2, dotprod466/2, dotprod467/2, dotprod468/2, dotprod469/2, dotprod470/2, dotprod471/2, dotprod472/2, dotprod473/2, dotprod474/2, dotprod475/2, dotprod476/2, dotprod477/2, dotprod478/2, dotprod479/2, dotprod480/2, dotprod481/2, dotprod482/2, dotprod483/2, dotprod484/2, dotprod485/2, dotprod486/2, dotprod487/2, dotprod488/2, dotprod489/2, dotprod490/2, dotprod491/2, dotprod492/2, dotprod493/2, dotprod494/2, dotprod495/2, dotprod496/2, dotprod497/2, dotprod498/2, dotprod499/2, dotprod500/2, dotprod501/2, dotprod502/2, dotprod503/2, dotprod504/2, dotprod505/2, dotprod506/2, dotprod507/2, dotprod508/2, dotprod509/2, dotprod510/2, dotprod511/2, dotprod512/2, dotprod513/2, dotprod514/2, dotprod515/2, dotprod516/2, dotprod517/2, dotprod518/2, dotprod519/2, dotprod520/2, dotprod521/2, dotprod522/2, dotprod523/2, dotprod524/2, dotprod525/2, dotprod526/2, dotprod527/2, dotprod528/2, dotprod529/2, dotprod530/2, dotprod531/2, dotprod532/2, dotprod533/2, dotprod534/2, dotprod535/2, dotprod536/2, dotprod537/2, dotprod538/2, dotprod539/2, dotprod540/2, dotprod541/2, dotprod542/2, dotprod543/2, dotprod544/2, dotprod545/2, dotprod546/2, dotprod547/2, dotprod548/2, dotprod549/2, dotprod550/2, dotprod551/2, dotprod552/2, dotprod553/2, dotprod554/2, dotprod555/2, dotprod556/2, dotprod557/2, dotprod558/2, dotprod559/2, dotprod560/2, dotprod561/2, dotprod562/2, dotprod563/2, dotprod564/2, dotprod565/2, dotprod566/2, dotprod567/2, dotprod568/2, dotprod569/2, dotprod570/2, dotprod571/2, dotprod572/2, dotprod573/2, dotprod574/2, dotprod575/2, dotprod576/2, dotprod577/2, dotprod578/2, dotprod579/2, dotprod580/2, dotprod581/2, dotprod582/2, dotprod583/2, dotprod584/2, dotprod585/2, dotprod586/2, dotprod587/2, dotprod588/2, dotprod589/2, dotprod590/2, dotprod591/2, dotprod592/2, dotprod593/2, dotprod594/2, dotprod595/2, dotprod596/2, dotprod597/2, dotprod598/2, dotprod599/2, dotprod600/2, dotprod601/2, dotprod602/2, dotprod603/2, dotprod604/2, dotprod605/2, dotprod606/2, dotprod607/2, dotprod608/2, dotprod609/2, dotprod610/2, dotprod611/2, dotprod612/2, dotprod613/2, dotprod614/2, dotprod615/2, dotprod616/2, dotprod617/2, dotprod618/2, dotprod619/2, dotprod620/2, dotprod621/2, dotprod622/2, dotprod623/2, dotprod624/2, dotprod625/2, dotprod626/2, dotprod627/2, dotprod628/2, dotprod629/2, dotprod630/2, dotprod631/2, dotprod632/2, dotprod633/2, dotprod634/2, dotprod635/2, dotprod636/2, dotprod637/2, dotprod638/2, dotprod639/2, dotprod640/2, dotprod641/2, dotprod642/2, dotprod643/2, dotprod644/2, dotprod645/2, dotprod646/2, dotprod647/2, dotprod648/2, dotprod649/2, dotprod650/2, dotprod651/2, dotprod652/2, dotprod653/2, dotprod654/2, dotprod655/2, dotprod656/2, dotprod657/2, dotprod658/2, dotprod659/2, dotprod660/2, dotprod661/2, dotprod662/2, dotprod663/2, dotprod664/2, dotprod665/2, dotprod666/2, dotprod667/2, dotprod668/2, dotprod669/2, dotprod670/2, dotprod671/2, dotprod672/2, dotprod673/2, dotprod674/2, dotprod675/2, dotprod676/2, dotprod677/2, dotprod678/2, dotprod679/2, dotprod680/2, dotprod681/2, dotprod682/2, dotprod683/2, dotprod684/2, dotprod685/2, dotprod686/2, dotprod687/2, dotprod688/2, dotprod689/2, dotprod690/2, dotprod691/2, dotprod692/2, dotprod693/2, dotprod694/2, dotprod695/2, dotprod696/2, dotprod697/2, dotprod698/2, dotprod699/2, dotprod700/2, dotprod701/2, dotprod702/2, dotprod703/2, dotprod704/2, dotprod705/2, dotprod706/2, dotprod707/2, dotprod708/2, dotprod709/2, dotprod710/2, dotprod711/2, dotprod712/2, dotprod713/2, dotprod714/2, dotprod715/2, dotprod716/2, dotprod717/2, dotprod718/2, dotprod719/2, dotprod720/2, dotprod721/2, dotprod722/2, dotprod723/2, dotprod724/2, dotprod725/2, dotprod726/2, dotprod727/2, dotprod728/2, dotprod729/2, dotprod730/2, dotprod731/2, dotprod732/2, dotprod733/2, dotprod734/2, dotprod735/2, dotprod736/2, dotprod737/2, dotprod738/2, dotprod739/2, dotprod740/2, dotprod741/2, dotprod742/2, dotprod743/2, dotprod744/2, dotprod745/2, dotprod746/2, dotprod747/2, dotprod748/2, dotprod749/2, dotprod750/2, dotprod751/2, dotprod752/2, dotprod753/2, dotprod754/2, dotprod755/2, dotprod756/2, dotprod757/2, dotprod758/2, dotprod759/2, dotprod760/2, dotprod761/2, dotprod762/2, dotprod763/2, dotprod764/2, dotprod765/2, dotprod766/2, dotprod767/2, dotprod768/2, dotprod769/2, dotprod770/2, dotprod771/2, dotprod772/2, dotprod773/2, dotprod774/2, dotprod775/2, dotprod776/2, dotprod777/2, dotprod778/2, dotprod779/2, dotprod780/2, dotprod781/2, dotprod782/2, dotprod783/2, dotprod784/2, dotprod785/2, dotprod786/2, dotprod787/2, dotprod788/2, dotprod789/2, dotprod790/2, dotprod791/2, dotprod792/2, dotprod793/2, dotprod794/2, dotprod795/2, dotprod796/2, dotprod797/2, dotprod798/2, dotprod799/2, dotprod800/2, dotprod801/2, dotprod802/2, dotprod803/2, dotprod804/2, dotprod805/2, dotprod806/2, dotprod807/2, dotprod808/2, dotprod809/2, dotprod810/2, dotprod811/2, dotprod812/2, dotprod813/2, dotprod814/2, dotprod815/2, dotprod816/2, dotprod817/2, dotprod818/2, dotprod819/2, dotprod820/2, dotprod821/2, dotprod822/2, dotprod823/2, dotprod824/2, dotprod825/2, dotprod826/2, dotprod827/2, dotprod828/2, dotprod829/2, dotprod830/2, dotprod831/2, dotprod832/2, dotprod833/2, dotprod834/2, dotprod835/2, dotprod836/2, dotprod837/2, dotprod838/2, dotprod839/2, dotprod840/2, dotprod841/2, dotprod842/2, dotprod843/2, dotprod844/2, dotprod845/2, dotprod846/2, dotprod847/2, dotprod848/2, dotprod849/2, dotprod850/2, dotprod851/2, dotprod852/2, dotprod853/2, dotprod854/2, dotprod855/2, dotprod856/2, dotprod857/2, dotprod858/2, dotprod859/2, dotprod860/2, dotprod861/2, dotprod862/2, dotprod863/2, dotprod864/2, dotprod865/2, dotprod866/2, dotprod867/2, dotprod868/2, dotprod869/2, dotprod870/2, dotprod871/2, dotprod872/2, dotprod873/2, dotprod874/2, dotprod875/2, dotprod876/2, dotprod877/2, dotprod878/2, dotprod879/2, dotprod880/2, dotprod881/2, dotprod882/2, dotprod883/2, dotprod884/2, dotprod885/2, dotprod886/2, dotprod887/2, dotprod888/2, dotprod889/2, dotprod890/2, dotprod891/2, dotprod892/2, dotprod893/2, dotprod894/2, dotprod895/2, dotprod896/2, dotprod897/2, dotprod898/2, dotprod899/2, dotprod900/2, dotprod901/2, dotprod902/2, dotprod903/2, dotprod904/2, dotprod905/2, dotprod906/2, dotprod907/2, dotprod908/2, dotprod909/2, dotprod910/2, dotprod911/2, dotprod912/2, dotprod913/2, dotprod914/2, dotprod915/2, dotprod916/2, dotprod917/2, dotprod918/2, dotprod919/2, dotprod920/2, dotprod921/2, dotprod922/2, dotprod923/2, dotprod924/2, dotprod925/2, dotprod926/2, dotprod927/2, dotprod928/2, dotprod929/2, dotprod930/2, dotprod931/2, dotprod932/2, dotprod933/2, dotprod934/2, dotprod935/2, dotprod936/2, dotprod937/2, dotprod938/2, dotprod939/2, dotprod940/2, dotprod941/2, dotprod942/2, dotprod943/2, dotprod944/2, dotprod945/2, dotprod946/2, dotprod947/2, dotprod948/2, dotprod949/2, dotprod950/2, dotprod951/2, dotprod952/2, dotprod953/2, dotprod954/2, dotprod955/2, dotprod956/2, dotprod957/2, dotprod958/2, dotprod959/2, dotprod960/2, dotprod961/2, dotprod962/2, dotprod963/2, dotprod964/2, dotprod965/2, dotprod966/2, dotprod967/2, dotprod968/2, dotprod969/2, dotprod970/2, dotprod971/2, dotprod972/2, dotprod973/2, dotprod974/2, dotprod975/2, dotprod976/2, dotprod977/2, dotprod978/2, dotprod979/2, dotprod980/2, dotprod981/2, dotprod982/2, dotprod983/2, dotprod984/2, dotprod985/2, dotprod986/2, dotprod987/2, dotprod988/2, dotprod989/2, dotprod990/2, dotprod991/2, dotprod992/2, dotprod993/2, dotprod994/2, dotprod995/2, dotprod996/2, dotprod997/2, dotprod998/2, dotprod999/2, dotprod1000/2, dotprod1001/2
  dotprod1/1 -> Mux/1
  "IW{2,1}(2,:)'"/1 -> dotprod2/1
  dotprod2/1 -> Mux/2
  "IW{2,1}(3,:)'"/1 -> dotprod3/1
  dotprod3/1 -> Mux/3
  "IW{2,1}(4,:)'"/1 -> dotprod4/1
  dotprod4/1 -> Mux/4
  "IW{2,1}(5,:)'"/1 -> dotprod5/1
  dotprod5/1 -> Mux/5
  "IW{2,1}(6,:)'"/1 -> dotprod6/1
  dotprod6/1 -> Mux/6
  "IW{2,1}(7,:)'"/1 -> dotprod7/1
  dotprod7/1 -> Mux/7
  "IW{2,1}(8,:)'"/1 -> dotprod8/1
  dotprod8/1 -> Mux/8
  "IW{2,1}(9,:)'"/1 -> dotprod9/1
  dotprod9/1 -> Mux/9
  "IW{2,1}(10,:)'"/1 -> dotprod10/1
  dotprod10/1 -> Mux/10
  "IW{2,1}(11,:)'"/1 -> dotprod11/1
  dotprod11/1 -> Mux/11
  "IW{2,1}(12,:)'"/1 -> dotprod12/1
  dotprod12/1 -> Mux/12
  "IW{2,1}(13,:)'"/1 -> dotprod13/1
  dotprod13/1 -> Mux/13
  "IW{2,1}(14,:)'"/1 -> dotprod14/1
  dotprod14/1 -> Mux/14
  "IW{2,1}(15,:)'"/1 -> dotprod15/1
  dotprod15/1 -> Mux/15
  "IW{2,1}(16,:)'"/1 -> dotprod16/1
  dotprod16/1 -> Mux/16
  "IW{2,1}(17,:)'"/1 -> dotprod17/1
  dotprod17/1 -> Mux/17
  "IW{2,1}(18,:)'"/1 -> dotprod18/1
  dotprod18/1 -> Mux/18
  "IW{2,1}(19,:)'"/1 -> dotprod19/1
  dotprod19/1 -> Mux/19
  "IW{2,1}(20,:)'"/1 -> dotprod20/1
  dotprod20/1 -> Mux/20
  "IW{2,1}(21,:)'"/1 -> dotprod21/1
  dotprod21/1 -> Mux/21
  "IW{2,1}(22,:)'"/1 -> dotprod22/1
  dotprod22/1 -> Mux/22
  "IW{2,1}(23,:)'"/1 -> dotprod23/1
  dotprod23/1 -> Mux/23
  "IW{2,1}(24,:)'"/1 -> dotprod24/1
  dotprod24/1 -> Mux/24
  "IW{2,1}(25,:)'"/1 -> dotprod25/1
  dotprod25/1 -> Mux/25
  "IW{2,1}(26,:)'"/1 -> dotprod26/1
  dotprod26/1 -> Mux/26
  "IW{2,1}(27,:)'"/1 -> dotprod27/1
  dotprod27/1 -> Mux/27
  "IW{2,1}(28,:)'"/1 -> dotprod28/1
  dotprod28/1 -> Mux/28
  "IW{2,1}(29,:)'"/1 -> dotprod29/1
  dotprod29/1 -> Mux/29
  "IW{2,1}(30,:)'"/1 -> dotprod30/1
  dotprod30/1 -> Mux/30
  "IW{2,1}(31,:)'"/1 -> dotprod31/1
  dotprod31/1 -> Mux/31
  "IW{2,1}(32,:)'"/1 -> dotprod32/1
  dotprod32/1 -> Mux/32
  "IW{2,1}(33,:)'"/1 -> dotprod33/1
  dotprod33/1 -> Mux/33
  "IW{2,1}(34,:)'"/1 -> dotprod34/1
  dotprod34/1 -> Mux/34
  "IW{2,1}(35,:)'"/1 -> dotprod35/1
  dotprod35/1 -> Mux/35
  "IW{2,1}(36,:)'"/1 -> dotprod36/1
  dotprod36/1 -> Mux/36
  "IW{2,1}(37,:)'"/1 -> dotprod37/1
  dotprod37/1 -> Mux/37
  "IW{2,1}(38,:)'"/1 -> dotprod38/1
  dotprod38/1 -> Mux/38
  "IW{2,1}(39,:)'"/1 -> dotprod39/1
  dotprod39/1 -> Mux/39
  "IW{2,1}(40,:)'"/1 -> dotprod40/1
  dotprod40/1 -> Mux/40
  "IW{2,1}(41,:)'"/1 -> dotprod41/1
  dotprod41/1 -> Mux/41
  "IW{2,1}(42,:)'"/1 -> dotprod42/1
  dotprod42/1 -> Mux/42
  "IW{2,1}(43,:)'"/1 -> dotprod43/1
  dotprod43/1 -> Mux/43
  "IW{2,1}(44,:)'"/1 -> dotprod44/1
  dotprod44/1 -> Mux/44
  "IW{2,1}(45,:)'"/1 -> dotprod45/1
  dotprod45/1 -> Mux/45
  "IW{2,1}(46,:)'"/1 -> dotprod46/1
  dotprod46/1 -> Mux/46
  "IW{2,1}(47,:)'"/1 -> dotprod47/1
  dotprod47/1 -> Mux/47
  "IW{2,1}(48,:)'"/1 -> dotprod48/1
  dotprod48/1 -> Mux/48
  "IW{2,1}(49,:)'"/1 -> dotprod49/1
  dotprod49/1 -> Mux/49
  "IW{2,1}(50,:)'"/1 -> dotprod50/1
  dotprod50/1 -> Mux/50
  "IW{2,1}(51,:)'"/1 -> dotprod51/1
  dotprod51/1 -> Mux/51
  "IW{2,1}(52,:)'"/1 -> dotprod52/1
  dotprod52/1 -> Mux/52
  "IW{2,1}(53,:)'"/1 -> dotprod53/1
  dotprod53/1 -> Mux/53
  "IW{2,1}(54,:)'"/1 -> dotprod54/1
  dotprod54/1 -> Mux/54
  "IW{2,1}(55,:)'"/1 -> dotprod55/1
  dotprod55/1 -> Mux/55
  "IW{2,1}(56,:)'"/1 -> dotprod56/1
  dotprod56/1 -> Mux/56
  "IW{2,1}(57,:)'"/1 -> dotprod57/1
  dotprod57/1 -> Mux/57
  "IW{2,1}(58,:)'"/1 -> dotprod58/1
  dotprod58/1 -> Mux/58
  "IW{2,1}(59,:)'"/1 -> dotprod59/1
  dotprod59/1 -> Mux/59
  "IW{2,1}(60,:)'"/1 -> dotprod60/1
  dotprod60/1 -> Mux/60
  "IW{2,1}(61,:)'"/1 -> dotprod61/1
  dotprod61/1 -> Mux/61
  "IW{2,1}(62,:)'"/1 -> dotprod62/1
  dotprod62/1 -> Mux/62
  "IW{2,1}(63,:)'"/1 -> dotprod63/1
  dotprod63/1 -> Mux/63
  "IW{2,1}(64,:)'"/1 -> dotprod64/1
  dotprod64/1 -> Mux/64
  "IW{2,1}(65,:)'"/1 -> dotprod65/1
  dotprod65/1 -> Mux/65
  "IW{2,1}(66,:)'"/1 -> dotprod66/1
  dotprod66/1 -> Mux/66
  "IW{2,1}(67,:)'"/1 -> dotprod67/1
  dotprod67/1 -> Mux/67
  "IW{2,1}(68,:)'"/1 -> dotprod68/1
  dotprod68/1 -> Mux/68
  "IW{2,1}(69,:)'"/1 -> dotprod69/1
  dotprod69/1 -> Mux/69
  "IW{2,1}(70,:)'"/1 -> dotprod70/1
  dotprod70/1 -> Mux/70
  "IW{2,1}(71,:)'"/1 -> dotprod71/1
  dotprod71/1 -> Mux/71
  "IW{2,1}(72,:)'"/1 -> dotprod72/1
  dotprod72/1 -> Mux/72
  "IW{2,1}(73,:)'"/1 -> dotprod73/1
  dotprod73/1 -> Mux/73
  "IW{2,1}(74,:)'"/1 -> dotprod74/1
  dotprod74/1 -> Mux/74
  "IW{2,1}(75,:)'"/1 -> dotprod75/1
  dotprod75/1 -> Mux/75
  "IW{2,1}(76,:)'"/1 -> dotprod76/1
  dotprod76/1 -> Mux/76
  "IW{2,1}(77,:)'"/1 -> dotprod77/1
  dotprod77/1 -> Mux/77
  "IW{2,1}(78,:)'"/1 -> dotprod78/1
  dotprod78/1 -> Mux/78
  "IW{2,1}(79,:)'"/1 -> dotprod79/1
  dotprod79/1 -> Mux/79
  "IW{2,1}(80,:)'"/1 -> dotprod80/1
  dotprod80/1 -> Mux/80
  "IW{2,1}(81,:)'"/1 -> dotprod81/1
  dotprod81/1 -> Mux/81
  "IW{2,1}(82,:)'"/1 -> dotprod82/1
  dotprod82/1 -> Mux/82
  "IW{2,1}(83,:)'"/1 -> dotprod83/1
  dotprod83/1 -> Mux/83
  "IW{2,1}(84,:)'"/1 -> dotprod84/1
  dotprod84/1 -> Mux/84
  "IW{2,1}(85,:)'"/1 -> dotprod85/1
  dotprod85/1 -> Mux/85
  "IW{2,1}(86,:)'"/1 -> dotprod86/1
  dotprod86/1 -> Mux/86
  "IW{2,1}(87,:)'"/1 -> dotprod87/1
  dotprod87/1 -> Mux/87
  "IW{2,1}(88,:)'"/1 -> dotprod88/1
  dotprod88/1 -> Mux/88
  "IW{2,1}(89,:)'"/1 -> dotprod89/1
  dotprod89/1 -> Mux/89
  "IW{2,1}(90,:)'"/1 -> dotprod90/1
  dotprod90/1 -> Mux/90
  "IW{2,1}(91,:)'"/1 -> dotprod91/1
  dotprod91/1 -> Mux/91
  "IW{2,1}(92,:)'"/1 -> dotprod92/1
  dotprod92/1 -> Mux/92
  "IW{2,1}(93,:)'"/1 -> dotprod93/1
  dotprod93/1 -> Mux/93
  "IW{2,1}(94,:)'"/1 -> dotprod94/1
  dotprod94/1 -> Mux/94
  "IW{2,1}(95,:)'"/1 -> dotprod95/1
  dotprod95/1 -> Mux/95
  "IW{2,1}(96,:)'"/1 -> dotprod96/1
  dotprod96/1 -> Mux/96
  "IW{2,1}(97,:)'"/1 -> dotprod97/1
  dotprod97/1 -> Mux/97
  "IW{2,1}(98,:)'"/1 -> dotprod98/1
  dotprod98/1 -> Mux/98
  "IW{2,1}(99,:)'"/1 -> dotprod99/1
  dotprod99/1 -> Mux/99
  "IW{2,1}(100,:)'"/1 -> dotprod100/1
  dotprod100/1 -> Mux/100
  "IW{2,1}(101,:)'"/1 -> dotprod101/1
  dotprod101/1 -> Mux/101
  "IW{2,1}(102,:)'"/1 -> dotprod102/1
  dotprod102/1 -> Mux/102
  "IW{2,1}(103,:)'"/1 -> dotprod103/1
  dotprod103/1 -> Mux/103
  "IW{2,1}(104,:)'"/1 -> dotprod104/1
  dotprod104/1 -> Mux/104
  "IW{2,1}(105,:)'"/1 -> dotprod105/1
  dotprod105/1 -> Mux/105
  "IW{2,1}(106,:)'"/1 -> dotprod106/1
  dotprod106/1 -> Mux/106
  "IW{2,1}(107,:)'"/1 -> dotprod107/1
  dotprod107/1 -> Mux/107
  "IW{2,1}(108,:)'"/1 -> dotprod108/1
  dotprod108/1 -> Mux/108
  "IW{2,1}(109,:)'"/1 -> dotprod109/1
  dotprod109/1 -> Mux/109
  "IW{2,1}(110,:)'"/1 -> dotprod110/1
  dotprod110/1 -> Mux/110
  "IW{2,1}(111,:)'"/1 -> dotprod111/1
  dotprod111/1 -> Mux/111
  "IW{2,1}(112,:)'"/1 -> dotprod112/1
  dotprod112/1 -> Mux/112
  "IW{2,1}(113,:)'"/1 -> dotprod113/1
  dotprod113/1 -> Mux/113
  "IW{2,1}(114,:)'"/1 -> dotprod114/1
  dotprod114/1 -> Mux/114
  "IW{2,1}(115,:)'"/1 -> dotprod115/1
  dotprod115/1 -> Mux/115
  "IW{2,1}(116,:)'"/1 -> dotprod116/1
  dotprod116/1 -> Mux/116
  "IW{2,1}(117,:)'"/1 -> dotprod117/1
  dotprod117/1 -> Mux/117
  "IW{2,1}(118,:)'"/1 -> dotprod118/1
  dotprod118/1 -> Mux/118
  "IW{2,1}(119,:)'"/1 -> dotprod119/1
  dotprod119/1 -> Mux/119
  "IW{2,1}(120,:)'"/1 -> dotprod120/1
  dotprod120/1 -> Mux/120
  "IW{2,1}(121,:)'"/1 -> dotprod121/1
  dotprod121/1 -> Mux/121
  "IW{2,1}(122,:)'"/1 -> dotprod122/1
  dotprod122/1 -> Mux/122
  "IW{2,1}(123,:)'"/1 -> dotprod123/1
  dotprod123/1 -> Mux/123
  "IW{2,1}(124,:)'"/1 -> dotprod124/1
  dotprod124/1 -> Mux/124
  "IW{2,1}(125,:)'"/1 -> dotprod125/1
  dotprod125/1 -> Mux/125
  "IW{2,1}(126,:)'"/1 -> dotprod126/1
  dotprod126/1 -> Mux/126
  "IW{2,1}(127,:)'"/1 -> dotprod127/1
  dotprod127/1 -> Mux/127
  "IW{2,1}(128,:)'"/1 -> dotprod128/1
  dotprod128/1 -> Mux/128
  "IW{2,1}(129,:)'"/1 -> dotprod129/1
  dotprod129/1 -> Mux/129
  "IW{2,1}(130,:)'"/1 -> dotprod130/1
  dotprod130/1 -> Mux/130
  "IW{2,1}(131,:)'"/1 -> dotprod131/1
  dotprod131/1 -> Mux/131
  "IW{2,1}(132,:)'"/1 -> dotprod132/1
  dotprod132/1 -> Mux/132
  "IW{2,1}(133,:)'"/1 -> dotprod133/1
  dotprod133/1 -> Mux/133
  "IW{2,1}(134,:)'"/1 -> dotprod134/1
  dotprod134/1 -> Mux/134
  "IW{2,1}(135,:)'"/1 -> dotprod135/1
  dotprod135/1 -> Mux/135
  "IW{2,1}(136,:)'"/1 -> dotprod136/1
  dotprod136/1 -> Mux/136
  "IW{2,1}(137,:)'"/1 -> dotprod137/1
  dotprod137/1 -> Mux/137
  "IW{2,1}(138,:)'"/1 -> dotprod138/1
  dotprod138/1 -> Mux/138
  "IW{2,1}(139,:)'"/1 -> dotprod139/1
  dotprod139/1 -> Mux/139
  "IW{2,1}(140,:)'"/1 -> dotprod140/1
  dotprod140/1 -> Mux/140
  "IW{2,1}(141,:)'"/1 -> dotprod141/1
  dotprod141/1 -> Mux/141
  "IW{2,1}(142,:)'"/1 -> dotprod142/1
  dotprod142/1 -> Mux/142
  "IW{2,1}(143,:)'"/1 -> dotprod143/1
  dotprod143/1 -> Mux/143
  "IW{2,1}(144,:)'"/1 -> dotprod144/1
  dotprod144/1 -> Mux/144
  "IW{2,1}(145,:)'"/1 -> dotprod145/1
  dotprod145/1 -> Mux/145
  "IW{2,1}(146,:)'"/1 -> dotprod146/1
  dotprod146/1 -> Mux/146
  "IW{2,1}(147,:)'"/1 -> dotprod147/1
  dotprod147/1 -> Mux/147
  "IW{2,1}(148,:)'"/1 -> dotprod148/1
  dotprod148/1 -> Mux/148
  "IW{2,1}(149,:)'"/1 -> dotprod149/1
  dotprod149/1 -> Mux/149
  "IW{2,1}(150,:)'"/1 -> dotprod150/1
  dotprod150/1 -> Mux/150
  "IW{2,1}(151,:)'"/1 -> dotprod151/1
  dotprod151/1 -> Mux/151
  "IW{2,1}(152,:)'"/1 -> dotprod152/1
  dotprod152/1 -> Mux/152
  "IW{2,1}(153,:)'"/1 -> dotprod153/1
  dotprod153/1 -> Mux/153
  "IW{2,1}(154,:)'"/1 -> dotprod154/1
  dotprod154/1 -> Mux/154
  "IW{2,1}(155,:)'"/1 -> dotprod155/1
  dotprod155/1 -> Mux/155
  "IW{2,1}(156,:)'"/1 -> dotprod156/1
  dotprod156/1 -> Mux/156
  "IW{2,1}(157,:)'"/1 -> dotprod157/1
  dotprod157/1 -> Mux/157
  "IW{2,1}(158,:)'"/1 -> dotprod158/1
  dotprod158/1 -> Mux/158
  "IW{2,1}(159,:)'"/1 -> dotprod159/1
  dotprod159/1 -> Mux/159
  "IW{2,1}(160,:)'"/1 -> dotprod160/1
  dotprod160/1 -> Mux/160
  "IW{2,1}(161,:)'"/1 -> dotprod161/1
  dotprod161/1 -> Mux/161
  "IW{2,1}(162,:)'"/1 -> dotprod162/1
  dotprod162/1 -> Mux/162
  "IW{2,1}(163,:)'"/1 -> dotprod163/1
  dotprod163/1 -> Mux/163
  "IW{2,1}(164,:)'"/1 -> dotprod164/1
  dotprod164/1 -> Mux/164
  "IW{2,1}(165,:)'"/1 -> dotprod165/1
  dotprod165/1 -> Mux/165
  "IW{2,1}(166,:)'"/1 -> dotprod166/1
  dotprod166/1 -> Mux/166
  "IW{2,1}(167,:)'"/1 -> dotprod167/1
  dotprod167/1 -> Mux/167
  "IW{2,1}(168,:)'"/1 -> dotprod168/1
  dotprod168/1 -> Mux/168
  "IW{2,1}(169,:)'"/1 -> dotprod169/1
  dotprod169/1 -> Mux/169
  "IW{2,1}(170,:)'"/1 -> dotprod170/1
  dotprod170/1 -> Mux/170
  "IW{2,1}(171,:)'"/1 -> dotprod171/1
  dotprod171/1 -> Mux/171
  "IW{2,1}(172,:)'"/1 -> dotprod172/1
  dotprod172/1 -> Mux/172
  "IW{2,1}(173,:)'"/1 -> dotprod173/1
  dotprod173/1 -> Mux/173
  "IW{2,1}(174,:)'"/1 -> dotprod174/1
  dotprod174/1 -> Mux/174
  "IW{2,1}(175,:)'"/1 -> dotprod175/1
  dotprod175/1 -> Mux/175
  "IW{2,1}(176,:)'"/1 -> dotprod176/1
  dotprod176/1 -> Mux/176
  "IW{2,1}(177,:)'"/1 -> dotprod177/1
  dotprod177/1 -> Mux/177
  "IW{2,1}(178,:)'"/1 -> dotprod178/1
  dotprod178/1 -> Mux/178
  "IW{2,1}(179,:)'"/1 -> dotprod179/1
  dotprod179/1 -> Mux/179
  "IW{2,1}(180,:)'"/1 -> dotprod180/1
  dotprod180/1 -> Mux/180
  "IW{2,1}(181,:)'"/1 -> dotprod181/1
  dotprod181/1 -> Mux/181
  "IW{2,1}(182,:)'"/1 -> dotprod182/1
  dotprod182/1 -> Mux/182
  "IW{2,1}(183,:)'"/1 -> dotprod183/1
  dotprod183/1 -> Mux/183
  "IW{2,1}(184,:)'"/1 -> dotprod184/1
  dotprod184/1 -> Mux/184
  "IW{2,1}(185,:)'"/1 -> dotprod185/1
  dotprod185/1 -> Mux/185
  "IW{2,1}(186,:)'"/1 -> dotprod186/1
  dotprod186/1 -> Mux/186
  "IW{2,1}(187,:)'"/1 -> dotprod187/1
  dotprod187/1 -> Mux/187
  "IW{2,1}(188,:)'"/1 -> dotprod188/1
  dotprod188/1 -> Mux/188
  "IW{2,1}(189,:)'"/1 -> dotprod189/1
  dotprod189/1 -> Mux/189
  "IW{2,1}(190,:)'"/1 -> dotprod190/1
  dotprod190/1 -> Mux/190
  "IW{2,1}(191,:)'"/1 -> dotprod191/1
  dotprod191/1 -> Mux/191
  "IW{2,1}(192,:)'"/1 -> dotprod192/1
  dotprod192/1 -> Mux/192
  "IW{2,1}(193,:)'"/1 -> dotprod193/1
  dotprod193/1 -> Mux/193
  "IW{2,1}(194,:)'"/1 -> dotprod194/1
  dotprod194/1 -> Mux/194
  "IW{2,1}(195,:)'"/1 -> dotprod195/1
  dotprod195/1 -> Mux/195
  "IW{2,1}(196,:)'"/1 -> dotprod196/1
  dotprod196/1 -> Mux/196
  "IW{2,1}(197,:)'"/1 -> dotprod197/1
  dotprod197/1 -> Mux/197
  "IW{2,1}(198,:)'"/1 -> dotprod198/1
  dotprod198/1 -> Mux/198
  "IW{2,1}(199,:)'"/1 -> dotprod199/1
  dotprod199/1 -> Mux/199
  "IW{2,1}(200,:)'"/1 -> dotprod200/1
  dotprod200/1 -> Mux/200
  "IW{2,1}(201,:)'"/1 -> dotprod201/1
  dotprod201/1 -> Mux/201
  "IW{2,1}(202,:)'"/1 -> dotprod202/1
  dotprod202/1 -> Mux/202
  "IW{2,1}(203,:)'"/1 -> dotprod203/1
  dotprod203/1 -> Mux/203
  "IW{2,1}(204,:)'"/1 -> dotprod204/1
  dotprod204/1 -> Mux/204
  "IW{2,1}(205,:)'"/1 -> dotprod205/1
  dotprod205/1 -> Mux/205
  "IW{2,1}(206,:)'"/1 -> dotprod206/1
  dotprod206/1 -> Mux/206
  "IW{2,1}(207,:)'"/1 -> dotprod207/1
  dotprod207/1 -> Mux/207
  "IW{2,1}(208,:)'"/1 -> dotprod208/1
  dotprod208/1 -> Mux/208
  "IW{2,1}(209,:)'"/1 -> dotprod209/1
  dotprod209/1 -> Mux/209
  "IW{2,1}(210,:)'"/1 -> dotprod210/1
  dotprod210/1 -> Mux/210
  "IW{2,1}(211,:)'"/1 -> dotprod211/1
  dotprod211/1 -> Mux/211
  "IW{2,1}(212,:)'"/1 -> dotprod212/1
  dotprod212/1 -> Mux/212
  "IW{2,1}(213,:)'"/1 -> dotprod213/1
  dotprod213/1 -> Mux/213
  "IW{2,1}(214,:)'"/1 -> dotprod214/1
  dotprod214/1 -> Mux/214
  "IW{2,1}(215,:)'"/1 -> dotprod215/1
  dotprod215/1 -> Mux/215
  "IW{2,1}(216,:)'"/1 -> dotprod216/1
  dotprod216/1 -> Mux/216
  "IW{2,1}(217,:)'"/1 -> dotprod217/1
  dotprod217/1 -> Mux/217
  "IW{2,1}(218,:)'"/1 -> dotprod218/1
  dotprod218/1 -> Mux/218
  "IW{2,1}(219,:)'"/1 -> dotprod219/1
  dotprod219/1 -> Mux/219
  "IW{2,1}(220,:)'"/1 -> dotprod220/1
  dotprod220/1 -> Mux/220
  "IW{2,1}(221,:)'"/1 -> dotprod221/1
  dotprod221/1 -> Mux/221
  "IW{2,1}(222,:)'"/1 -> dotprod222/1
  dotprod222/1 -> Mux/222
  "IW{2,1}(223,:)'"/1 -> dotprod223/1
  dotprod223/1 -> Mux/223
  "IW{2,1}(224,:)'"/1 -> dotprod224/1
  dotprod224/1 -> Mux/224
  "IW{2,1}(225,:)'"/1 -> dotprod225/1
  dotprod225/1 -> Mux/225
  "IW{2,1}(226,:)'"/1 -> dotprod226/1
  dotprod226/1 -> Mux/226
  "IW{2,1}(227,:)'"/1 -> dotprod227/1
  dotprod227/1 -> Mux/227
  "IW{2,1}(228,:)'"/1 -> dotprod228/1
  dotprod228/1 -> Mux/228
  "IW{2,1}(229,:)'"/1 -> dotprod229/1
  dotprod229/1 -> Mux/229
  "IW{2,1}(230,:)'"/1 -> dotprod230/1
  dotprod230/1 -> Mux/230
  "IW{2,1}(231,:)'"/1 -> dotprod231/1
  dotprod231/1 -> Mux/231
  "IW{2,1}(232,:)'"/1 -> dotprod232/1
  dotprod232/1 -> Mux/232
  "IW{2,1}(233,:)'"/1 -> dotprod233/1
  dotprod233/1 -> Mux/233
  "IW{2,1}(234,:)'"/1 -> dotprod234/1
  dotprod234/1 -> Mux/234
  "IW{2,1}(235,:)'"/1 -> dotprod235/1
  dotprod235/1 -> Mux/235
  "IW{2,1}(236,:)'"/1 -> dotprod236/1
  dotprod236/1 -> Mux/236
  "IW{2,1}(237,:)'"/1 -> dotprod237/1
  dotprod237/1 -> Mux/237
  "IW{2,1}(238,:)'"/1 -> dotprod238/1
  dotprod238/1 -> Mux/238
  "IW{2,1}(239,:)'"/1 -> dotprod239/1
  dotprod239/1 -> Mux/239
  "IW{2,1}(240,:)'"/1 -> dotprod240/1
  dotprod240/1 -> Mux/240
  "IW{2,1}(241,:)'"/1 -> dotprod241/1
  dotprod241/1 -> Mux/241
  "IW{2,1}(242,:)'"/1 -> dotprod242/1
  dotprod242/1 -> Mux/242
  "IW{2,1}(243,:)'"/1 -> dotprod243/1
  dotprod243/1 -> Mux/243
  "IW{2,1}(244,:)'"/1 -> dotprod244/1
  dotprod244/1 -> Mux/244
  "IW{2,1}(245,:)'"/1 -> dotprod245/1
  dotprod245/1 -> Mux/245
  "IW{2,1}(246,:)'"/1 -> dotprod246/1
  dotprod246/1 -> Mux/246
  "IW{2,1}(247,:)'"/1 -> dotprod247/1
  dotprod247/1 -> Mux/247
  "IW{2,1}(248,:)'"/1 -> dotprod248/1
  dotprod248/1 -> Mux/248
  "IW{2,1}(249,:)'"/1 -> dotprod249/1
  dotprod249/1 -> Mux/249
  "IW{2,1}(250,:)'"/1 -> dotprod250/1
  dotprod250/1 -> Mux/250
  "IW{2,1}(251,:)'"/1 -> dotprod251/1
  dotprod251/1 -> Mux/251
  "IW{2,1}(252,:)'"/1 -> dotprod252/1
  dotprod252/1 -> Mux/252
  "IW{2,1}(253,:)'"/1 -> dotprod253/1
  dotprod253/1 -> Mux/253
  "IW{2,1}(254,:)'"/1 -> dotprod254/1
  dotprod254/1 -> Mux/254
  "IW{2,1}(255,:)'"/1 -> dotprod255/1
  dotprod255/1 -> Mux/255
  "IW{2,1}(256,:)'"/1 -> dotprod256/1
  dotprod256/1 -> Mux/256
  "IW{2,1}(257,:)'"/1 -> dotprod257/1
  dotprod257/1 -> Mux/257
  "IW{2,1}(258,:)'"/1 -> dotprod258/1
  dotprod258/1 -> Mux/258
  "IW{2,1}(259,:)'"/1 -> dotprod259/1
  dotprod259/1 -> Mux/259
  "IW{2,1}(260,:)'"/1 -> dotprod260/1
  dotprod260/1 -> Mux/260
  "IW{2,1}(261,:)'"/1 -> dotprod261/1
  dotprod261/1 -> Mux/261
  "IW{2,1}(262,:)'"/1 -> dotprod262/1
  dotprod262/1 -> Mux/262
  "IW{2,1}(263,:)'"/1 -> dotprod263/1
  dotprod263/1 -> Mux/263
  "IW{2,1}(264,:)'"/1 -> dotprod264/1
  dotprod264/1 -> Mux/264
  "IW{2,1}(265,:)'"/1 -> dotprod265/1
  dotprod265/1 -> Mux/265
  "IW{2,1}(266,:)'"/1 -> dotprod266/1
  dotprod266/1 -> Mux/266
  "IW{2,1}(267,:)'"/1 -> dotprod267/1
  dotprod267/1 -> Mux/267
  "IW{2,1}(268,:)'"/1 -> dotprod268/1
  dotprod268/1 -> Mux/268
  "IW{2,1}(269,:)'"/1 -> dotprod269/1
  dotprod269/1 -> Mux/269
  "IW{2,1}(270,:)'"/1 -> dotprod270/1
  dotprod270/1 -> Mux/270
  "IW{2,1}(271,:)'"/1 -> dotprod271/1
  dotprod271/1 -> Mux/271
  "IW{2,1}(272,:)'"/1 -> dotprod272/1
  dotprod272/1 -> Mux/272
  "IW{2,1}(273,:)'"/1 -> dotprod273/1
  dotprod273/1 -> Mux/273
  "IW{2,1}(274,:)'"/1 -> dotprod274/1
  dotprod274/1 -> Mux/274
  "IW{2,1}(275,:)'"/1 -> dotprod275/1
  dotprod275/1 -> Mux/275
  "IW{2,1}(276,:)'"/1 -> dotprod276/1
  dotprod276/1 -> Mux/276
  "IW{2,1}(277,:)'"/1 -> dotprod277/1
  dotprod277/1 -> Mux/277
  "IW{2,1}(278,:)'"/1 -> dotprod278/1
  dotprod278/1 -> Mux/278
  "IW{2,1}(279,:)'"/1 -> dotprod279/1
  dotprod279/1 -> Mux/279
  "IW{2,1}(280,:)'"/1 -> dotprod280/1
  dotprod280/1 -> Mux/280
  "IW{2,1}(281,:)'"/1 -> dotprod281/1
  dotprod281/1 -> Mux/281
  "IW{2,1}(282,:)'"/1 -> dotprod282/1
  dotprod282/1 -> Mux/282
  "IW{2,1}(283,:)'"/1 -> dotprod283/1
  dotprod283/1 -> Mux/283
  "IW{2,1}(284,:)'"/1 -> dotprod284/1
  dotprod284/1 -> Mux/284
  "IW{2,1}(285,:)'"/1 -> dotprod285/1
  dotprod285/1 -> Mux/285
  "IW{2,1}(286,:)'"/1 -> dotprod286/1
  dotprod286/1 -> Mux/286
  "IW{2,1}(287,:)'"/1 -> dotprod287/1
  dotprod287/1 -> Mux/287
  "IW{2,1}(288,:)'"/1 -> dotprod288/1
  dotprod288/1 -> Mux/288
  "IW{2,1}(289,:)'"/1 -> dotprod289/1
  dotprod289/1 -> Mux/289
  "IW{2,1}(290,:)'"/1 -> dotprod290/1
  dotprod290/1 -> Mux/290
  "IW{2,1}(291,:)'"/1 -> dotprod291/1
  dotprod291/1 -> Mux/291
  "IW{2,1}(292,:)'"/1 -> dotprod292/1
  dotprod292/1 -> Mux/292
  "IW{2,1}(293,:)'"/1 -> dotprod293/1
  dotprod293/1 -> Mux/293
  "IW{2,1}(294,:)'"/1 -> dotprod294/1
  dotprod294/1 -> Mux/294
  "IW{2,1}(295,:)'"/1 -> dotprod295/1
  dotprod295/1 -> Mux/295
  "IW{2,1}(296,:)'"/1 -> dotprod296/1
  dotprod296/1 -> Mux/296
  "IW{2,1}(297,:)'"/1 -> dotprod297/1
  dotprod297/1 -> Mux/297
  "IW{2,1}(298,:)'"/1 -> dotprod298/1
  dotprod298/1 -> Mux/298
  "IW{2,1}(299,:)'"/1 -> dotprod299/1
  dotprod299/1 -> Mux/299
  "IW{2,1}(300,:)'"/1 -> dotprod300/1
  dotprod300/1 -> Mux/300
  "IW{2,1}(301,:)'"/1 -> dotprod301/1
  dotprod301/1 -> Mux/301
  "IW{2,1}(302,:)'"/1 -> dotprod302/1
  dotprod302/1 -> Mux/302
  "IW{2,1}(303,:)'"/1 -> dotprod303/1
  dotprod303/1 -> Mux/303
  "IW{2,1}(304,:)'"/1 -> dotprod304/1
  dotprod304/1 -> Mux/304
  "IW{2,1}(305,:)'"/1 -> dotprod305/1
  dotprod305/1 -> Mux/305
  "IW{2,1}(306,:)'"/1 -> dotprod306/1
  dotprod306/1 -> Mux/306
  "IW{2,1}(307,:)'"/1 -> dotprod307/1
  dotprod307/1 -> Mux/307
  "IW{2,1}(308,:)'"/1 -> dotprod308/1
  dotprod308/1 -> Mux/308
  "IW{2,1}(309,:)'"/1 -> dotprod309/1
  dotprod309/1 -> Mux/309
  "IW{2,1}(310,:)'"/1 -> dotprod310/1
  dotprod310/1 -> Mux/310
  "IW{2,1}(311,:)'"/1 -> dotprod311/1
  dotprod311/1 -> Mux/311
  "IW{2,1}(312,:)'"/1 -> dotprod312/1
  dotprod312/1 -> Mux/312
  "IW{2,1}(313,:)'"/1 -> dotprod313/1
  dotprod313/1 -> Mux/313
  "IW{2,1}(314,:)'"/1 -> dotprod314/1
  dotprod314/1 -> Mux/314
  "IW{2,1}(315,:)'"/1 -> dotprod315/1
  dotprod315/1 -> Mux/315
  "IW{2,1}(316,:)'"/1 -> dotprod316/1
  dotprod316/1 -> Mux/316
  "IW{2,1}(317,:)'"/1 -> dotprod317/1
  dotprod317/1 -> Mux/317
  "IW{2,1}(318,:)'"/1 -> dotprod318/1
  dotprod318/1 -> Mux/318
  "IW{2,1}(319,:)'"/1 -> dotprod319/1
  dotprod319/1 -> Mux/319
  "IW{2,1}(320,:)'"/1 -> dotprod320/1
  dotprod320/1 -> Mux/320
  "IW{2,1}(321,:)'"/1 -> dotprod321/1
  dotprod321/1 -> Mux/321
  "IW{2,1}(322,:)'"/1 -> dotprod322/1
  dotprod322/1 -> Mux/322
  "IW{2,1}(323,:)'"/1 -> dotprod323/1
  dotprod323/1 -> Mux/323
  "IW{2,1}(324,:)'"/1 -> dotprod324/1
  dotprod324/1 -> Mux/324
  "IW{2,1}(325,:)'"/1 -> dotprod325/1
  dotprod325/1 -> Mux/325
  "IW{2,1}(326,:)'"/1 -> dotprod326/1
  dotprod326/1 -> Mux/326
  "IW{2,1}(327,:)'"/1 -> dotprod327/1
  dotprod327/1 -> Mux/327
  "IW{2,1}(328,:)'"/1 -> dotprod328/1
  dotprod328/1 -> Mux/328
  "IW{2,1}(329,:)'"/1 -> dotprod329/1
  dotprod329/1 -> Mux/329
  "IW{2,1}(330,:)'"/1 -> dotprod330/1
  dotprod330/1 -> Mux/330
  "IW{2,1}(331,:)'"/1 -> dotprod331/1
  dotprod331/1 -> Mux/331
  "IW{2,1}(332,:)'"/1 -> dotprod332/1
  dotprod332/1 -> Mux/332
  "IW{2,1}(333,:)'"/1 -> dotprod333/1
  dotprod333/1 -> Mux/333
  "IW{2,1}(334,:)'"/1 -> dotprod334/1
  dotprod334/1 -> Mux/334
  "IW{2,1}(335,:)'"/1 -> dotprod335/1
  dotprod335/1 -> Mux/335
  "IW{2,1}(336,:)'"/1 -> dotprod336/1
  dotprod336/1 -> Mux/336
  "IW{2,1}(337,:)'"/1 -> dotprod337/1
  dotprod337/1 -> Mux/337
  "IW{2,1}(338,:)'"/1 -> dotprod338/1
  dotprod338/1 -> Mux/338
  "IW{2,1}(339,:)'"/1 -> dotprod339/1
  dotprod339/1 -> Mux/339
  "IW{2,1}(340,:)'"/1 -> dotprod340/1
  dotprod340/1 -> Mux/340
  "IW{2,1}(341,:)'"/1 -> dotprod341/1
  dotprod341/1 -> Mux/341
  "IW{2,1}(342,:)'"/1 -> dotprod342/1
  dotprod342/1 -> Mux/342
  "IW{2,1}(343,:)'"/1 -> dotprod343/1
  dotprod343/1 -> Mux/343
  "IW{2,1}(344,:)'"/1 -> dotprod344/1
  dotprod344/1 -> Mux/344
  "IW{2,1}(345,:)'"/1 -> dotprod345/1
  dotprod345/1 -> Mux/345
  "IW{2,1}(346,:)'"/1 -> dotprod346/1
  dotprod346/1 -> Mux/346
  "IW{2,1}(347,:)'"/1 -> dotprod347/1
  dotprod347/1 -> Mux/347
  "IW{2,1}(348,:)'"/1 -> dotprod348/1
  dotprod348/1 -> Mux/348
  "IW{2,1}(349,:)'"/1 -> dotprod349/1
  dotprod349/1 -> Mux/349
  "IW{2,1}(350,:)'"/1 -> dotprod350/1
  dotprod350/1 -> Mux/350
  "IW{2,1}(351,:)'"/1 -> dotprod351/1
  dotprod351/1 -> Mux/351
  "IW{2,1}(352,:)'"/1 -> dotprod352/1
  dotprod352/1 -> Mux/352
  "IW{2,1}(353,:)'"/1 -> dotprod353/1
  dotprod353/1 -> Mux/353
  "IW{2,1}(354,:)'"/1 -> dotprod354/1
  dotprod354/1 -> Mux/354
  "IW{2,1}(355,:)'"/1 -> dotprod355/1
  dotprod355/1 -> Mux/355
  "IW{2,1}(356,:)'"/1 -> dotprod356/1
  dotprod356/1 -> Mux/356
  "IW{2,1}(357,:)'"/1 -> dotprod357/1
  dotprod357/1 -> Mux/357
  "IW{2,1}(358,:)'"/1 -> dotprod358/1
  dotprod358/1 -> Mux/358
  "IW{2,1}(359,:)'"/1 -> dotprod359/1
  dotprod359/1 -> Mux/359
  "IW{2,1}(360,:)'"/1 -> dotprod360/1
  dotprod360/1 -> Mux/360
  "IW{2,1}(361,:)'"/1 -> dotprod361/1
  dotprod361/1 -> Mux/361
  "IW{2,1}(362,:)'"/1 -> dotprod362/1
  dotprod362/1 -> Mux/362
  "IW{2,1}(363,:)'"/1 -> dotprod363/1
  dotprod363/1 -> Mux/363
  "IW{2,1}(364,:)'"/1 -> dotprod364/1
  dotprod364/1 -> Mux/364
  "IW{2,1}(365,:)'"/1 -> dotprod365/1
  dotprod365/1 -> Mux/365
  "IW{2,1}(366,:)'"/1 -> dotprod366/1
  dotprod366/1 -> Mux/366
  "IW{2,1}(367,:)'"/1 -> dotprod367/1
  dotprod367/1 -> Mux/367
  "IW{2,1}(368,:)'"/1 -> dotprod368/1
  dotprod368/1 -> Mux/368
  "IW{2,1}(369,:)'"/1 -> dotprod369/1
  dotprod369/1 -> Mux/369
  "IW{2,1}(370,:)'"/1 -> dotprod370/1
  dotprod370/1 -> Mux/370
  "IW{2,1}(371,:)'"/1 -> dotprod371/1
  dotprod371/1 -> Mux/371
  "IW{2,1}(372,:)'"/1 -> dotprod372/1
  dotprod372/1 -> Mux/372
  "IW{2,1}(373,:)'"/1 -> dotprod373/1
  dotprod373/1 -> Mux/373
  "IW{2,1}(374,:)'"/1 -> dotprod374/1
  dotprod374/1 -> Mux/374
  "IW{2,1}(375,:)'"/1 -> dotprod375/1
  dotprod375/1 -> Mux/375
  "IW{2,1}(376,:)'"/1 -> dotprod376/1
  dotprod376/1 -> Mux/376
  "IW{2,1}(377,:)'"/1 -> dotprod377/1
  dotprod377/1 -> Mux/377
  "IW{2,1}(378,:)'"/1 -> dotprod378/1
  dotprod378/1 -> Mux/378
  "IW{2,1}(379,:)'"/1 -> dotprod379/1
  dotprod379/1 -> Mux/379
  "IW{2,1}(380,:)'"/1 -> dotprod380/1
  dotprod380/1 -> Mux/380
  "IW{2,1}(381,:)'"/1 -> dotprod381/1
  dotprod381/1 -> Mux/381
  "IW{2,1}(382,:)'"/1 -> dotprod382/1
  dotprod382/1 -> Mux/382
  "IW{2,1}(383,:)'"/1 -> dotprod383/1
  dotprod383/1 -> Mux/383
  "IW{2,1}(384,:)'"/1 -> dotprod384/1
  dotprod384/1 -> Mux/384
  "IW{2,1}(385,:)'"/1 -> dotprod385/1
  dotprod385/1 -> Mux/385
  "IW{2,1}(386,:)'"/1 -> dotprod386/1
  dotprod386/1 -> Mux/386
  "IW{2,1}(387,:)'"/1 -> dotprod387/1
  dotprod387/1 -> Mux/387
  "IW{2,1}(388,:)'"/1 -> dotprod388/1
  dotprod388/1 -> Mux/388
  "IW{2,1}(389,:)'"/1 -> dotprod389/1
  dotprod389/1 -> Mux/389
  "IW{2,1}(390,:)'"/1 -> dotprod390/1
  dotprod390/1 -> Mux/390
  "IW{2,1}(391,:)'"/1 -> dotprod391/1
  dotprod391/1 -> Mux/391
  "IW{2,1}(392,:)'"/1 -> dotprod392/1
  dotprod392/1 -> Mux/392
  "IW{2,1}(393,:)'"/1 -> dotprod393/1
  dotprod393/1 -> Mux/393
  "IW{2,1}(394,:)'"/1 -> dotprod394/1
  dotprod394/1 -> Mux/394
  "IW{2,1}(395,:)'"/1 -> dotprod395/1
  dotprod395/1 -> Mux/395
  "IW{2,1}(396,:)'"/1 -> dotprod396/1
  dotprod396/1 -> Mux/396
  "IW{2,1}(397,:)'"/1 -> dotprod397/1
  dotprod397/1 -> Mux/397
  "IW{2,1}(398,:)'"/1 -> dotprod398/1
  dotprod398/1 -> Mux/398
  "IW{2,1}(399,:)'"/1 -> dotprod399/1
  dotprod399/1 -> Mux/399
  "IW{2,1}(400,:)'"/1 -> dotprod400/1
  dotprod400/1 -> Mux/400
  "IW{2,1}(401,:)'"/1 -> dotprod401/1
  dotprod401/1 -> Mux/401
  "IW{2,1}(402,:)'"/1 -> dotprod402/1
  dotprod402/1 -> Mux/402
  "IW{2,1}(403,:)'"/1 -> dotprod403/1
  dotprod403/1 -> Mux/403
  "IW{2,1}(404,:)'"/1 -> dotprod404/1
  dotprod404/1 -> Mux/404
  "IW{2,1}(405,:)'"/1 -> dotprod405/1
  dotprod405/1 -> Mux/405
  "IW{2,1}(406,:)'"/1 -> dotprod406/1
  dotprod406/1 -> Mux/406
  "IW{2,1}(407,:)'"/1 -> dotprod407/1
  dotprod407/1 -> Mux/407
  "IW{2,1}(408,:)'"/1 -> dotprod408/1
  dotprod408/1 -> Mux/408
  "IW{2,1}(409,:)'"/1 -> dotprod409/1
  dotprod409/1 -> Mux/409
  "IW{2,1}(410,:)'"/1 -> dotprod410/1
  dotprod410/1 -> Mux/410
  "IW{2,1}(411,:)'"/1 -> dotprod411/1
  dotprod411/1 -> Mux/411
  "IW{2,1}(412,:)'"/1 -> dotprod412/1
  dotprod412/1 -> Mux/412
  "IW{2,1}(413,:)'"/1 -> dotprod413/1
  dotprod413/1 -> Mux/413
  "IW{2,1}(414,:)'"/1 -> dotprod414/1
  dotprod414/1 -> Mux/414
  "IW{2,1}(415,:)'"/1 -> dotprod415/1
  dotprod415/1 -> Mux/415
  "IW{2,1}(416,:)'"/1 -> dotprod416/1
  dotprod416/1 -> Mux/416
  "IW{2,1}(417,:)'"/1 -> dotprod417/1
  dotprod417/1 -> Mux/417
  "IW{2,1}(418,:)'"/1 -> dotprod418/1
  dotprod418/1 -> Mux/418
  "IW{2,1}(419,:)'"/1 -> dotprod419/1
  dotprod419/1 -> Mux/419
  "IW{2,1}(420,:)'"/1 -> dotprod420/1
  dotprod420/1 -> Mux/420
  "IW{2,1}(421,:)'"/1 -> dotprod421/1
  dotprod421/1 -> Mux/421
  "IW{2,1}(422,:)'"/1 -> dotprod422/1
  dotprod422/1 -> Mux/422
  "IW{2,1}(423,:)'"/1 -> dotprod423/1
  dotprod423/1 -> Mux/423
  "IW{2,1}(424,:)'"/1 -> dotprod424/1
  dotprod424/1 -> Mux/424
  "IW{2,1}(425,:)'"/1 -> dotprod425/1
  dotprod425/1 -> Mux/425
  "IW{2,1}(426,:)'"/1 -> dotprod426/1
  dotprod426/1 -> Mux/426
  "IW{2,1}(427,:)'"/1 -> dotprod427/1
  dotprod427/1 -> Mux/427
  "IW{2,1}(428,:)'"/1 -> dotprod428/1
  dotprod428/1 -> Mux/428
  "IW{2,1}(429,:)'"/1 -> dotprod429/1
  dotprod429/1 -> Mux/429
  "IW{2,1}(430,:)'"/1 -> dotprod430/1
  dotprod430/1 -> Mux/430
  "IW{2,1}(431,:)'"/1 -> dotprod431/1
  dotprod431/1 -> Mux/431
  "IW{2,1}(432,:)'"/1 -> dotprod432/1
  dotprod432/1 -> Mux/432
  "IW{2,1}(433,:)'"/1 -> dotprod433/1
  dotprod433/1 -> Mux/433
  "IW{2,1}(434,:)'"/1 -> dotprod434/1
  dotprod434/1 -> Mux/434
  "IW{2,1}(435,:)'"/1 -> dotprod435/1
  dotprod435/1 -> Mux/435
  "IW{2,1}(436,:)'"/1 -> dotprod436/1
  dotprod436/1 -> Mux/436
  "IW{2,1}(437,:)'"/1 -> dotprod437/1
  dotprod437/1 -> Mux/437
  "IW{2,1}(438,:)'"/1 -> dotprod438/1
  dotprod438/1 -> Mux/438
  "IW{2,1}(439,:)'"/1 -> dotprod439/1
  dotprod439/1 -> Mux/439
  "IW{2,1}(440,:)'"/1 -> dotprod440/1
  dotprod440/1 -> Mux/440
  "IW{2,1}(441,:)'"/1 -> dotprod441/1
  dotprod441/1 -> Mux/441
  "IW{2,1}(442,:)'"/1 -> dotprod442/1
  dotprod442/1 -> Mux/442
  "IW{2,1}(443,:)'"/1 -> dotprod443/1
  dotprod443/1 -> Mux/443
  "IW{2,1}(444,:)'"/1 -> dotprod444/1
  dotprod444/1 -> Mux/444
  "IW{2,1}(445,:)'"/1 -> dotprod445/1
  dotprod445/1 -> Mux/445
  "IW{2,1}(446,:)'"/1 -> dotprod446/1
  dotprod446/1 -> Mux/446
  "IW{2,1}(447,:)'"/1 -> dotprod447/1
  dotprod447/1 -> Mux/447
  "IW{2,1}(448,:)'"/1 -> dotprod448/1
  dotprod448/1 -> Mux/448
  "IW{2,1}(449,:)'"/1 -> dotprod449/1
  dotprod449/1 -> Mux/449
  "IW{2,1}(450,:)'"/1 -> dotprod450/1
  dotprod450/1 -> Mux/450
  "IW{2,1}(451,:)'"/1 -> dotprod451/1
  dotprod451/1 -> Mux/451
  "IW{2,1}(452,:)'"/1 -> dotprod452/1
  dotprod452/1 -> Mux/452
  "IW{2,1}(453,:)'"/1 -> dotprod453/1
  dotprod453/1 -> Mux/453
  "IW{2,1}(454,:)'"/1 -> dotprod454/1
  dotprod454/1 -> Mux/454
  "IW{2,1}(455,:)'"/1 -> dotprod455/1
  dotprod455/1 -> Mux/455
  "IW{2,1}(456,:)'"/1 -> dotprod456/1
  dotprod456/1 -> Mux/456
  "IW{2,1}(457,:)'"/1 -> dotprod457/1
  dotprod457/1 -> Mux/457
  "IW{2,1}(458,:)'"/1 -> dotprod458/1
  dotprod458/1 -> Mux/458
  "IW{2,1}(459,:)'"/1 -> dotprod459/1
  dotprod459/1 -> Mux/459
  "IW{2,1}(460,:)'"/1 -> dotprod460/1
  dotprod460/1 -> Mux/460
  "IW{2,1}(461,:)'"/1 -> dotprod461/1
  dotprod461/1 -> Mux/461
  "IW{2,1}(462,:)'"/1 -> dotprod462/1
  dotprod462/1 -> Mux/462
  "IW{2,1}(463,:)'"/1 -> dotprod463/1
  dotprod463/1 -> Mux/463
  "IW{2,1}(464,:)'"/1 -> dotprod464/1
  dotprod464/1 -> Mux/464
  "IW{2,1}(465,:)'"/1 -> dotprod465/1
  dotprod465/1 -> Mux/465
  "IW{2,1}(466,:)'"/1 -> dotprod466/1
  dotprod466/1 -> Mux/466
  "IW{2,1}(467,:)'"/1 -> dotprod467/1
  dotprod467/1 -> Mux/467
  "IW{2,1}(468,:)'"/1 -> dotprod468/1
  dotprod468/1 -> Mux/468
  "IW{2,1}(469,:)'"/1 -> dotprod469/1
  dotprod469/1 -> Mux/469
  "IW{2,1}(470,:)'"/1 -> dotprod470/1
  dotprod470/1 -> Mux/470
  "IW{2,1}(471,:)'"/1 -> dotprod471/1
  dotprod471/1 -> Mux/471
  "IW{2,1}(472,:)'"/1 -> dotprod472/1
  dotprod472/1 -> Mux/472
  "IW{2,1}(473,:)'"/1 -> dotprod473/1
  dotprod473/1 -> Mux/473
  "IW{2,1}(474,:)'"/1 -> dotprod474/1
  dotprod474/1 -> Mux/474
  "IW{2,1}(475,:)'"/1 -> dotprod475/1
  dotprod475/1 -> Mux/475
  "IW{2,1}(476,:)'"/1 -> dotprod476/1
  dotprod476/1 -> Mux/476
  "IW{2,1}(477,:)'"/1 -> dotprod477/1
  dotprod477/1 -> Mux/477
  "IW{2,1}(478,:)'"/1 -> dotprod478/1
  dotprod478/1 -> Mux/478
  "IW{2,1}(479,:)'"/1 -> dotprod479/1
  dotprod479/1 -> Mux/479
  "IW{2,1}(480,:)'"/1 -> dotprod480/1
  dotprod480/1 -> Mux/480
  "IW{2,1}(481,:)'"/1 -> dotprod481/1
  dotprod481/1 -> Mux/481
  "IW{2,1}(482,:)'"/1 -> dotprod482/1
  dotprod482/1 -> Mux/482
  "IW{2,1}(483,:)'"/1 -> dotprod483/1
  dotprod483/1 -> Mux/483
  "IW{2,1}(484,:)'"/1 -> dotprod484/1
  dotprod484/1 -> Mux/484
  "IW{2,1}(485,:)'"/1 -> dotprod485/1
  dotprod485/1 -> Mux/485
  "IW{2,1}(486,:)'"/1 -> dotprod486/1
  dotprod486/1 -> Mux/486
  "IW{2,1}(487,:)'"/1 -> dotprod487/1
  dotprod487/1 -> Mux/487
  "IW{2,1}(488,:)'"/1 -> dotprod488/1
  dotprod488/1 -> Mux/488
  "IW{2,1}(489,:)'"/1 -> dotprod489/1
  dotprod489/1 -> Mux/489
  "IW{2,1}(490,:)'"/1 -> dotprod490/1
  dotprod490/1 -> Mux/490
  "IW{2,1}(491,:)'"/1 -> dotprod491/1
  dotprod491/1 -> Mux/491
  "IW{2,1}(492,:)'"/1 -> dotprod492/1
  dotprod492/1 -> Mux/492
  "IW{2,1}(493,:)'"/1 -> dotprod493/1
  dotprod493/1 -> Mux/493
  "IW{2,1}(494,:)'"/1 -> dotprod494/1
  dotprod494/1 -> Mux/494
  "IW{2,1}(495,:)'"/1 -> dotprod495/1
  dotprod495/1 -> Mux/495
  "IW{2,1}(496,:)'"/1 -> dotprod496/1
  dotprod496/1 -> Mux/496
  "IW{2,1}(497,:)'"/1 -> dotprod497/1
  dotprod497/1 -> Mux/497
  "IW{2,1}(498,:)'"/1 -> dotprod498/1
  dotprod498/1 -> Mux/498
  "IW{2,1}(499,:)'"/1 -> dotprod499/1
  dotprod499/1 -> Mux/499
  "IW{2,1}(500,:)'"/1 -> dotprod500/1
  dotprod500/1 -> Mux/500
  "IW{2,1}(501,:)'"/1 -> dotprod501/1
  dotprod501/1 -> Mux/501
  "IW{2,1}(502,:)'"/1 -> dotprod502/1
  dotprod502/1 -> Mux/502
  "IW{2,1}(503,:)'"/1 -> dotprod503/1
  dotprod503/1 -> Mux/503
  "IW{2,1}(504,:)'"/1 -> dotprod504/1
  dotprod504/1 -> Mux/504
  "IW{2,1}(505,:)'"/1 -> dotprod505/1
  dotprod505/1 -> Mux/505
  "IW{2,1}(506,:)'"/1 -> dotprod506/1
  dotprod506/1 -> Mux/506
  "IW{2,1}(507,:)'"/1 -> dotprod507/1
  dotprod507/1 -> Mux/507
  "IW{2,1}(508,:)'"/1 -> dotprod508/1
  dotprod508/1 -> Mux/508
  "IW{2,1}(509,:)'"/1 -> dotprod509/1
  dotprod509/1 -> Mux/509
  "IW{2,1}(510,:)'"/1 -> dotprod510/1
  dotprod510/1 -> Mux/510
  "IW{2,1}(511,:)'"/1 -> dotprod511/1
  dotprod511/1 -> Mux/511
  "IW{2,1}(512,:)'"/1 -> dotprod512/1
  dotprod512/1 -> Mux/512
  "IW{2,1}(513,:)'"/1 -> dotprod513/1
  dotprod513/1 -> Mux/513
  "IW{2,1}(514,:)'"/1 -> dotprod514/1
  dotprod514/1 -> Mux/514
  "IW{2,1}(515,:)'"/1 -> dotprod515/1
  dotprod515/1 -> Mux/515
  "IW{2,1}(516,:)'"/1 -> dotprod516/1
  dotprod516/1 -> Mux/516
  "IW{2,1}(517,:)'"/1 -> dotprod517/1
  dotprod517/1 -> Mux/517
  "IW{2,1}(518,:)'"/1 -> dotprod518/1
  dotprod518/1 -> Mux/518
  "IW{2,1}(519,:)'"/1 -> dotprod519/1
  dotprod519/1 -> Mux/519
  "IW{2,1}(520,:)'"/1 -> dotprod520/1
  dotprod520/1 -> Mux/520
  "IW{2,1}(521,:)'"/1 -> dotprod521/1
  dotprod521/1 -> Mux/521
  "IW{2,1}(522,:)'"/1 -> dotprod522/1
  dotprod522/1 -> Mux/522
  "IW{2,1}(523,:)'"/1 -> dotprod523/1
  dotprod523/1 -> Mux/523
  "IW{2,1}(524,:)'"/1 -> dotprod524/1
  dotprod524/1 -> Mux/524
  "IW{2,1}(525,:)'"/1 -> dotprod525/1
  dotprod525/1 -> Mux/525
  "IW{2,1}(526,:)'"/1 -> dotprod526/1
  dotprod526/1 -> Mux/526
  "IW{2,1}(527,:)'"/1 -> dotprod527/1
  dotprod527/1 -> Mux/527
  "IW{2,1}(528,:)'"/1 -> dotprod528/1
  dotprod528/1 -> Mux/528
  "IW{2,1}(529,:)'"/1 -> dotprod529/1
  dotprod529/1 -> Mux/529
  "IW{2,1}(530,:)'"/1 -> dotprod530/1
  dotprod530/1 -> Mux/530
  "IW{2,1}(531,:)'"/1 -> dotprod531/1
  dotprod531/1 -> Mux/531
  "IW{2,1}(532,:)'"/1 -> dotprod532/1
  dotprod532/1 -> Mux/532
  "IW{2,1}(533,:)'"/1 -> dotprod533/1
  dotprod533/1 -> Mux/533
  "IW{2,1}(534,:)'"/1 -> dotprod534/1
  dotprod534/1 -> Mux/534
  "IW{2,1}(535,:)'"/1 -> dotprod535/1
  dotprod535/1 -> Mux/535
  "IW{2,1}(536,:)'"/1 -> dotprod536/1
  dotprod536/1 -> Mux/536
  "IW{2,1}(537,:)'"/1 -> dotprod537/1
  dotprod537/1 -> Mux/537
  "IW{2,1}(538,:)'"/1 -> dotprod538/1
  dotprod538/1 -> Mux/538
  "IW{2,1}(539,:)'"/1 -> dotprod539/1
  dotprod539/1 -> Mux/539
  "IW{2,1}(540,:)'"/1 -> dotprod540/1
  dotprod540/1 -> Mux/540
  "IW{2,1}(541,:)'"/1 -> dotprod541/1
  dotprod541/1 -> Mux/541
  "IW{2,1}(542,:)'"/1 -> dotprod542/1
  dotprod542/1 -> Mux/542
  "IW{2,1}(543,:)'"/1 -> dotprod543/1
  dotprod543/1 -> Mux/543
  "IW{2,1}(544,:)'"/1 -> dotprod544/1
  dotprod544/1 -> Mux/544
  "IW{2,1}(545,:)'"/1 -> dotprod545/1
  dotprod545/1 -> Mux/545
  "IW{2,1}(546,:)'"/1 -> dotprod546/1
  dotprod546/1 -> Mux/546
  "IW{2,1}(547,:)'"/1 -> dotprod547/1
  dotprod547/1 -> Mux/547
  "IW{2,1}(548,:)'"/1 -> dotprod548/1
  dotprod548/1 -> Mux/548
  "IW{2,1}(549,:)'"/1 -> dotprod549/1
  dotprod549/1 -> Mux/549
  "IW{2,1}(550,:)'"/1 -> dotprod550/1
  dotprod550/1 -> Mux/550
  "IW{2,1}(551,:)'"/1 -> dotprod551/1
  dotprod551/1 -> Mux/551
  "IW{2,1}(552,:)'"/1 -> dotprod552/1
  dotprod552/1 -> Mux/552
  "IW{2,1}(553,:)'"/1 -> dotprod553/1
  dotprod553/1 -> Mux/553
  "IW{2,1}(554,:)'"/1 -> dotprod554/1
  dotprod554/1 -> Mux/554
  "IW{2,1}(555,:)'"/1 -> dotprod555/1
  dotprod555/1 -> Mux/555
  "IW{2,1}(556,:)'"/1 -> dotprod556/1
  dotprod556/1 -> Mux/556
  "IW{2,1}(557,:)'"/1 -> dotprod557/1
  dotprod557/1 -> Mux/557
  "IW{2,1}(558,:)'"/1 -> dotprod558/1
  dotprod558/1 -> Mux/558
  "IW{2,1}(559,:)'"/1 -> dotprod559/1
  dotprod559/1 -> Mux/559
  "IW{2,1}(560,:)'"/1 -> dotprod560/1
  dotprod560/1 -> Mux/560
  "IW{2,1}(561,:)'"/1 -> dotprod561/1
  dotprod561/1 -> Mux/561
  "IW{2,1}(562,:)'"/1 -> dotprod562/1
  dotprod562/1 -> Mux/562
  "IW{2,1}(563,:)'"/1 -> dotprod563/1
  dotprod563/1 -> Mux/563
  "IW{2,1}(564,:)'"/1 -> dotprod564/1
  dotprod564/1 -> Mux/564
  "IW{2,1}(565,:)'"/1 -> dotprod565/1
  dotprod565/1 -> Mux/565
  "IW{2,1}(566,:)'"/1 -> dotprod566/1
  dotprod566/1 -> Mux/566
  "IW{2,1}(567,:)'"/1 -> dotprod567/1
  dotprod567/1 -> Mux/567
  "IW{2,1}(568,:)'"/1 -> dotprod568/1
  dotprod568/1 -> Mux/568
  "IW{2,1}(569,:)'"/1 -> dotprod569/1
  dotprod569/1 -> Mux/569
  "IW{2,1}(570,:)'"/1 -> dotprod570/1
  dotprod570/1 -> Mux/570
  "IW{2,1}(571,:)'"/1 -> dotprod571/1
  dotprod571/1 -> Mux/571
  "IW{2,1}(572,:)'"/1 -> dotprod572/1
  dotprod572/1 -> Mux/572
  "IW{2,1}(573,:)'"/1 -> dotprod573/1
  dotprod573/1 -> Mux/573
  "IW{2,1}(574,:)'"/1 -> dotprod574/1
  dotprod574/1 -> Mux/574
  "IW{2,1}(575,:)'"/1 -> dotprod575/1
  dotprod575/1 -> Mux/575
  "IW{2,1}(576,:)'"/1 -> dotprod576/1
  dotprod576/1 -> Mux/576
  "IW{2,1}(577,:)'"/1 -> dotprod577/1
  dotprod577/1 -> Mux/577
  "IW{2,1}(578,:)'"/1 -> dotprod578/1
  dotprod578/1 -> Mux/578
  "IW{2,1}(579,:)'"/1 -> dotprod579/1
  dotprod579/1 -> Mux/579
  "IW{2,1}(580,:)'"/1 -> dotprod580/1
  dotprod580/1 -> Mux/580
  "IW{2,1}(581,:)'"/1 -> dotprod581/1
  dotprod581/1 -> Mux/581
  "IW{2,1}(582,:)'"/1 -> dotprod582/1
  dotprod582/1 -> Mux/582
  "IW{2,1}(583,:)'"/1 -> dotprod583/1
  dotprod583/1 -> Mux/583
  "IW{2,1}(584,:)'"/1 -> dotprod584/1
  dotprod584/1 -> Mux/584
  "IW{2,1}(585,:)'"/1 -> dotprod585/1
  dotprod585/1 -> Mux/585
  "IW{2,1}(586,:)'"/1 -> dotprod586/1
  dotprod586/1 -> Mux/586
  "IW{2,1}(587,:)'"/1 -> dotprod587/1
  dotprod587/1 -> Mux/587
  "IW{2,1}(588,:)'"/1 -> dotprod588/1
  dotprod588/1 -> Mux/588
  "IW{2,1}(589,:)'"/1 -> dotprod589/1
  dotprod589/1 -> Mux/589
  "IW{2,1}(590,:)'"/1 -> dotprod590/1
  dotprod590/1 -> Mux/590
  "IW{2,1}(591,:)'"/1 -> dotprod591/1
  dotprod591/1 -> Mux/591
  "IW{2,1}(592,:)'"/1 -> dotprod592/1
  dotprod592/1 -> Mux/592
  "IW{2,1}(593,:)'"/1 -> dotprod593/1
  dotprod593/1 -> Mux/593
  "IW{2,1}(594,:)'"/1 -> dotprod594/1
  dotprod594/1 -> Mux/594
  "IW{2,1}(595,:)'"/1 -> dotprod595/1
  dotprod595/1 -> Mux/595
  "IW{2,1}(596,:)'"/1 -> dotprod596/1
  dotprod596/1 -> Mux/596
  "IW{2,1}(597,:)'"/1 -> dotprod597/1
  dotprod597/1 -> Mux/597
  "IW{2,1}(598,:)'"/1 -> dotprod598/1
  dotprod598/1 -> Mux/598
  "IW{2,1}(599,:)'"/1 -> dotprod599/1
  dotprod599/1 -> Mux/599
  "IW{2,1}(600,:)'"/1 -> dotprod600/1
  dotprod600/1 -> Mux/600
  "IW{2,1}(601,:)'"/1 -> dotprod601/1
  dotprod601/1 -> Mux/601
  "IW{2,1}(602,:)'"/1 -> dotprod602/1
  dotprod602/1 -> Mux/602
  "IW{2,1}(603,:)'"/1 -> dotprod603/1
  dotprod603/1 -> Mux/603
  "IW{2,1}(604,:)'"/1 -> dotprod604/1
  dotprod604/1 -> Mux/604
  "IW{2,1}(605,:)'"/1 -> dotprod605/1
  dotprod605/1 -> Mux/605
  "IW{2,1}(606,:)'"/1 -> dotprod606/1
  dotprod606/1 -> Mux/606
  "IW{2,1}(607,:)'"/1 -> dotprod607/1
  dotprod607/1 -> Mux/607
  "IW{2,1}(608,:)'"/1 -> dotprod608/1
  dotprod608/1 -> Mux/608
  "IW{2,1}(609,:)'"/1 -> dotprod609/1
  dotprod609/1 -> Mux/609
  "IW{2,1}(610,:)'"/1 -> dotprod610/1
  dotprod610/1 -> Mux/610
  "IW{2,1}(611,:)'"/1 -> dotprod611/1
  dotprod611/1 -> Mux/611
  "IW{2,1}(612,:)'"/1 -> dotprod612/1
  dotprod612/1 -> Mux/612
  "IW{2,1}(613,:)'"/1 -> dotprod613/1
  dotprod613/1 -> Mux/613
  "IW{2,1}(614,:)'"/1 -> dotprod614/1
  dotprod614/1 -> Mux/614
  "IW{2,1}(615,:)'"/1 -> dotprod615/1
  dotprod615/1 -> Mux/615
  "IW{2,1}(616,:)'"/1 -> dotprod616/1
  dotprod616/1 -> Mux/616
  "IW{2,1}(617,:)'"/1 -> dotprod617/1
  dotprod617/1 -> Mux/617
  "IW{2,1}(618,:)'"/1 -> dotprod618/1
  dotprod618/1 -> Mux/618
  "IW{2,1}(619,:)'"/1 -> dotprod619/1
  dotprod619/1 -> Mux/619
  "IW{2,1}(620,:)'"/1 -> dotprod620/1
  dotprod620/1 -> Mux/620
  "IW{2,1}(621,:)'"/1 -> dotprod621/1
  dotprod621/1 -> Mux/621
  "IW{2,1}(622,:)'"/1 -> dotprod622/1
  dotprod622/1 -> Mux/622
  "IW{2,1}(623,:)'"/1 -> dotprod623/1
  dotprod623/1 -> Mux/623
  "IW{2,1}(624,:)'"/1 -> dotprod624/1
  dotprod624/1 -> Mux/624
  "IW{2,1}(625,:)'"/1 -> dotprod625/1
  dotprod625/1 -> Mux/625
  "IW{2,1}(626,:)'"/1 -> dotprod626/1
  dotprod626/1 -> Mux/626
  "IW{2,1}(627,:)'"/1 -> dotprod627/1
  dotprod627/1 -> Mux/627
  "IW{2,1}(628,:)'"/1 -> dotprod628/1
  dotprod628/1 -> Mux/628
  "IW{2,1}(629,:)'"/1 -> dotprod629/1
  dotprod629/1 -> Mux/629
  "IW{2,1}(630,:)'"/1 -> dotprod630/1
  dotprod630/1 -> Mux/630
  "IW{2,1}(631,:)'"/1 -> dotprod631/1
  dotprod631/1 -> Mux/631
  "IW{2,1}(632,:)'"/1 -> dotprod632/1
  dotprod632/1 -> Mux/632
  "IW{2,1}(633,:)'"/1 -> dotprod633/1
  dotprod633/1 -> Mux/633
  "IW{2,1}(634,:)'"/1 -> dotprod634/1
  dotprod634/1 -> Mux/634
  "IW{2,1}(635,:)'"/1 -> dotprod635/1
  dotprod635/1 -> Mux/635
  "IW{2,1}(636,:)'"/1 -> dotprod636/1
  dotprod636/1 -> Mux/636
  "IW{2,1}(637,:)'"/1 -> dotprod637/1
  dotprod637/1 -> Mux/637
  "IW{2,1}(638,:)'"/1 -> dotprod638/1
  dotprod638/1 -> Mux/638
  "IW{2,1}(639,:)'"/1 -> dotprod639/1
  dotprod639/1 -> Mux/639
  "IW{2,1}(640,:)'"/1 -> dotprod640/1
  dotprod640/1 -> Mux/640
  "IW{2,1}(641,:)'"/1 -> dotprod641/1
  dotprod641/1 -> Mux/641
  "IW{2,1}(642,:)'"/1 -> dotprod642/1
  dotprod642/1 -> Mux/642
  "IW{2,1}(643,:)'"/1 -> dotprod643/1
  dotprod643/1 -> Mux/643
  "IW{2,1}(644,:)'"/1 -> dotprod644/1
  dotprod644/1 -> Mux/644
  "IW{2,1}(645,:)'"/1 -> dotprod645/1
  dotprod645/1 -> Mux/645
  "IW{2,1}(646,:)'"/1 -> dotprod646/1
  dotprod646/1 -> Mux/646
  "IW{2,1}(647,:)'"/1 -> dotprod647/1
  dotprod647/1 -> Mux/647
  "IW{2,1}(648,:)'"/1 -> dotprod648/1
  dotprod648/1 -> Mux/648
  "IW{2,1}(649,:)'"/1 -> dotprod649/1
  dotprod649/1 -> Mux/649
  "IW{2,1}(650,:)'"/1 -> dotprod650/1
  dotprod650/1 -> Mux/650
  "IW{2,1}(651,:)'"/1 -> dotprod651/1
  dotprod651/1 -> Mux/651
  "IW{2,1}(652,:)'"/1 -> dotprod652/1
  dotprod652/1 -> Mux/652
  "IW{2,1}(653,:)'"/1 -> dotprod653/1
  dotprod653/1 -> Mux/653
  "IW{2,1}(654,:)'"/1 -> dotprod654/1
  dotprod654/1 -> Mux/654
  "IW{2,1}(655,:)'"/1 -> dotprod655/1
  dotprod655/1 -> Mux/655
  "IW{2,1}(656,:)'"/1 -> dotprod656/1
  dotprod656/1 -> Mux/656
  "IW{2,1}(657,:)'"/1 -> dotprod657/1
  dotprod657/1 -> Mux/657
  "IW{2,1}(658,:)'"/1 -> dotprod658/1
  dotprod658/1 -> Mux/658
  "IW{2,1}(659,:)'"/1 -> dotprod659/1
  dotprod659/1 -> Mux/659
  "IW{2,1}(660,:)'"/1 -> dotprod660/1
  dotprod660/1 -> Mux/660
  "IW{2,1}(661,:)'"/1 -> dotprod661/1
  dotprod661/1 -> Mux/661
  "IW{2,1}(662,:)'"/1 -> dotprod662/1
  dotprod662/1 -> Mux/662
  "IW{2,1}(663,:)'"/1 -> dotprod663/1
  dotprod663/1 -> Mux/663
  "IW{2,1}(664,:)'"/1 -> dotprod664/1
  dotprod664/1 -> Mux/664
  "IW{2,1}(665,:)'"/1 -> dotprod665/1
  dotprod665/1 -> Mux/665
  "IW{2,1}(666,:)'"/1 -> dotprod666/1
  dotprod666/1 -> Mux/666
  "IW{2,1}(667,:)'"/1 -> dotprod667/1
  dotprod667/1 -> Mux/667
  "IW{2,1}(668,:)'"/1 -> dotprod668/1
  dotprod668/1 -> Mux/668
  "IW{2,1}(669,:)'"/1 -> dotprod669/1
  dotprod669/1 -> Mux/669
  "IW{2,1}(670,:)'"/1 -> dotprod670/1
  dotprod670/1 -> Mux/670
  "IW{2,1}(671,:)'"/1 -> dotprod671/1
  dotprod671/1 -> Mux/671
  "IW{2,1}(672,:)'"/1 -> dotprod672/1
  dotprod672/1 -> Mux/672
  "IW{2,1}(673,:)'"/1 -> dotprod673/1
  dotprod673/1 -> Mux/673
  "IW{2,1}(674,:)'"/1 -> dotprod674/1
  dotprod674/1 -> Mux/674
  "IW{2,1}(675,:)'"/1 -> dotprod675/1
  dotprod675/1 -> Mux/675
  "IW{2,1}(676,:)'"/1 -> dotprod676/1
  dotprod676/1 -> Mux/676
  "IW{2,1}(677,:)'"/1 -> dotprod677/1
  dotprod677/1 -> Mux/677
  "IW{2,1}(678,:)'"/1 -> dotprod678/1
  dotprod678/1 -> Mux/678
  "IW{2,1}(679,:)'"/1 -> dotprod679/1
  dotprod679/1 -> Mux/679
  "IW{2,1}(680,:)'"/1 -> dotprod680/1
  dotprod680/1 -> Mux/680
  "IW{2,1}(681,:)'"/1 -> dotprod681/1
  dotprod681/1 -> Mux/681
  "IW{2,1}(682,:)'"/1 -> dotprod682/1
  dotprod682/1 -> Mux/682
  "IW{2,1}(683,:)'"/1 -> dotprod683/1
  dotprod683/1 -> Mux/683
  "IW{2,1}(684,:)'"/1 -> dotprod684/1
  dotprod684/1 -> Mux/684
  "IW{2,1}(685,:)'"/1 -> dotprod685/1
  dotprod685/1 -> Mux/685
  "IW{2,1}(686,:)'"/1 -> dotprod686/1
  dotprod686/1 -> Mux/686
  "IW{2,1}(687,:)'"/1 -> dotprod687/1
  dotprod687/1 -> Mux/687
  "IW{2,1}(688,:)'"/1 -> dotprod688/1
  dotprod688/1 -> Mux/688
  "IW{2,1}(689,:)'"/1 -> dotprod689/1
  dotprod689/1 -> Mux/689
  "IW{2,1}(690,:)'"/1 -> dotprod690/1
  dotprod690/1 -> Mux/690
  "IW{2,1}(691,:)'"/1 -> dotprod691/1
  dotprod691/1 -> Mux/691
  "IW{2,1}(692,:)'"/1 -> dotprod692/1
  dotprod692/1 -> Mux/692
  "IW{2,1}(693,:)'"/1 -> dotprod693/1
  dotprod693/1 -> Mux/693
  "IW{2,1}(694,:)'"/1 -> dotprod694/1
  dotprod694/1 -> Mux/694
  "IW{2,1}(695,:)'"/1 -> dotprod695/1
  dotprod695/1 -> Mux/695
  "IW{2,1}(696,:)'"/1 -> dotprod696/1
  dotprod696/1 -> Mux/696
  "IW{2,1}(697,:)'"/1 -> dotprod697/1
  dotprod697/1 -> Mux/697
  "IW{2,1}(698,:)'"/1 -> dotprod698/1
  dotprod698/1 -> Mux/698
  "IW{2,1}(699,:)'"/1 -> dotprod699/1
  dotprod699/1 -> Mux/699
  "IW{2,1}(700,:)'"/1 -> dotprod700/1
  dotprod700/1 -> Mux/700
  "IW{2,1}(701,:)'"/1 -> dotprod701/1
  dotprod701/1 -> Mux/701
  "IW{2,1}(702,:)'"/1 -> dotprod702/1
  dotprod702/1 -> Mux/702
  "IW{2,1}(703,:)'"/1 -> dotprod703/1
  dotprod703/1 -> Mux/703
  "IW{2,1}(704,:)'"/1 -> dotprod704/1
  dotprod704/1 -> Mux/704
  "IW{2,1}(705,:)'"/1 -> dotprod705/1
  dotprod705/1 -> Mux/705
  "IW{2,1}(706,:)'"/1 -> dotprod706/1
  dotprod706/1 -> Mux/706
  "IW{2,1}(707,:)'"/1 -> dotprod707/1
  dotprod707/1 -> Mux/707
  "IW{2,1}(708,:)'"/1 -> dotprod708/1
  dotprod708/1 -> Mux/708
  "IW{2,1}(709,:)'"/1 -> dotprod709/1
  dotprod709/1 -> Mux/709
  "IW{2,1}(710,:)'"/1 -> dotprod710/1
  dotprod710/1 -> Mux/710
  "IW{2,1}(711,:)'"/1 -> dotprod711/1
  dotprod711/1 -> Mux/711
  "IW{2,1}(712,:)'"/1 -> dotprod712/1
  dotprod712/1 -> Mux/712
  "IW{2,1}(713,:)'"/1 -> dotprod713/1
  dotprod713/1 -> Mux/713
  "IW{2,1}(714,:)'"/1 -> dotprod714/1
  dotprod714/1 -> Mux/714
  "IW{2,1}(715,:)'"/1 -> dotprod715/1
  dotprod715/1 -> Mux/715
  "IW{2,1}(716,:)'"/1 -> dotprod716/1
  dotprod716/1 -> Mux/716
  "IW{2,1}(717,:)'"/1 -> dotprod717/1
  dotprod717/1 -> Mux/717
  "IW{2,1}(718,:)'"/1 -> dotprod718/1
  dotprod718/1 -> Mux/718
  "IW{2,1}(719,:)'"/1 -> dotprod719/1
  dotprod719/1 -> Mux/719
  "IW{2,1}(720,:)'"/1 -> dotprod720/1
  dotprod720/1 -> Mux/720
  "IW{2,1}(721,:)'"/1 -> dotprod721/1
  dotprod721/1 -> Mux/721
  "IW{2,1}(722,:)'"/1 -> dotprod722/1
  dotprod722/1 -> Mux/722
  "IW{2,1}(723,:)'"/1 -> dotprod723/1
  dotprod723/1 -> Mux/723
  "IW{2,1}(724,:)'"/1 -> dotprod724/1
  dotprod724/1 -> Mux/724
  "IW{2,1}(725,:)'"/1 -> dotprod725/1
  dotprod725/1 -> Mux/725
  "IW{2,1}(726,:)'"/1 -> dotprod726/1
  dotprod726/1 -> Mux/726
  "IW{2,1}(727,:)'"/1 -> dotprod727/1
  dotprod727/1 -> Mux/727
  "IW{2,1}(728,:)'"/1 -> dotprod728/1
  dotprod728/1 -> Mux/728
  "IW{2,1}(729,:)'"/1 -> dotprod729/1
  dotprod729/1 -> Mux/729
  "IW{2,1}(730,:)'"/1 -> dotprod730/1
  dotprod730/1 -> Mux/730
  "IW{2,1}(731,:)'"/1 -> dotprod731/1
  dotprod731/1 -> Mux/731
  "IW{2,1}(732,:)'"/1 -> dotprod732/1
  dotprod732/1 -> Mux/732
  "IW{2,1}(733,:)'"/1 -> dotprod733/1
  dotprod733/1 -> Mux/733
  "IW{2,1}(734,:)'"/1 -> dotprod734/1
  dotprod734/1 -> Mux/734
  "IW{2,1}(735,:)'"/1 -> dotprod735/1
  dotprod735/1 -> Mux/735
  "IW{2,1}(736,:)'"/1 -> dotprod736/1
  dotprod736/1 -> Mux/736
  "IW{2,1}(737,:)'"/1 -> dotprod737/1
  dotprod737/1 -> Mux/737
  "IW{2,1}(738,:)'"/1 -> dotprod738/1
  dotprod738/1 -> Mux/738
  "IW{2,1}(739,:)'"/1 -> dotprod739/1
  dotprod739/1 -> Mux/739
  "IW{2,1}(740,:)'"/1 -> dotprod740/1
  dotprod740/1 -> Mux/740
  "IW{2,1}(741,:)'"/1 -> dotprod741/1
  dotprod741/1 -> Mux/741
  "IW{2,1}(742,:)'"/1 -> dotprod742/1
  dotprod742/1 -> Mux/742
  "IW{2,1}(743,:)'"/1 -> dotprod743/1
  dotprod743/1 -> Mux/743
  "IW{2,1}(744,:)'"/1 -> dotprod744/1
  dotprod744/1 -> Mux/744
  "IW{2,1}(745,:)'"/1 -> dotprod745/1
  dotprod745/1 -> Mux/745
  "IW{2,1}(746,:)'"/1 -> dotprod746/1
  dotprod746/1 -> Mux/746
  "IW{2,1}(747,:)'"/1 -> dotprod747/1
  dotprod747/1 -> Mux/747
  "IW{2,1}(748,:)'"/1 -> dotprod748/1
  dotprod748/1 -> Mux/748
  "IW{2,1}(749,:)'"/1 -> dotprod749/1
  dotprod749/1 -> Mux/749
  "IW{2,1}(750,:)'"/1 -> dotprod750/1
  dotprod750/1 -> Mux/750
  "IW{2,1}(751,:)'"/1 -> dotprod751/1
  dotprod751/1 -> Mux/751
  "IW{2,1}(752,:)'"/1 -> dotprod752/1
  dotprod752/1 -> Mux/752
  "IW{2,1}(753,:)'"/1 -> dotprod753/1
  dotprod753/1 -> Mux/753
  "IW{2,1}(754,:)'"/1 -> dotprod754/1
  dotprod754/1 -> Mux/754
  "IW{2,1}(755,:)'"/1 -> dotprod755/1
  dotprod755/1 -> Mux/755
  "IW{2,1}(756,:)'"/1 -> dotprod756/1
  dotprod756/1 -> Mux/756
  "IW{2,1}(757,:)'"/1 -> dotprod757/1
  dotprod757/1 -> Mux/757
  "IW{2,1}(758,:)'"/1 -> dotprod758/1
  dotprod758/1 -> Mux/758
  "IW{2,1}(759,:)'"/1 -> dotprod759/1
  dotprod759/1 -> Mux/759
  "IW{2,1}(760,:)'"/1 -> dotprod760/1
  dotprod760/1 -> Mux/760
  "IW{2,1}(761,:)'"/1 -> dotprod761/1
  dotprod761/1 -> Mux/761
  "IW{2,1}(762,:)'"/1 -> dotprod762/1
  dotprod762/1 -> Mux/762
  "IW{2,1}(763,:)'"/1 -> dotprod763/1
  dotprod763/1 -> Mux/763
  "IW{2,1}(764,:)'"/1 -> dotprod764/1
  dotprod764/1 -> Mux/764
  "IW{2,1}(765,:)'"/1 -> dotprod765/1
  dotprod765/1 -> Mux/765
  "IW{2,1}(766,:)'"/1 -> dotprod766/1
  dotprod766/1 -> Mux/766
  "IW{2,1}(767,:)'"/1 -> dotprod767/1
  dotprod767/1 -> Mux/767
  "IW{2,1}(768,:)'"/1 -> dotprod768/1
  dotprod768/1 -> Mux/768
  "IW{2,1}(769,:)'"/1 -> dotprod769/1
  dotprod769/1 -> Mux/769
  "IW{2,1}(770,:)'"/1 -> dotprod770/1
  dotprod770/1 -> Mux/770
  "IW{2,1}(771,:)'"/1 -> dotprod771/1
  dotprod771/1 -> Mux/771
  "IW{2,1}(772,:)'"/1 -> dotprod772/1
  dotprod772/1 -> Mux/772
  "IW{2,1}(773,:)'"/1 -> dotprod773/1
  dotprod773/1 -> Mux/773
  "IW{2,1}(774,:)'"/1 -> dotprod774/1
  dotprod774/1 -> Mux/774
  "IW{2,1}(775,:)'"/1 -> dotprod775/1
  dotprod775/1 -> Mux/775
  "IW{2,1}(776,:)'"/1 -> dotprod776/1
  dotprod776/1 -> Mux/776
  "IW{2,1}(777,:)'"/1 -> dotprod777/1
  dotprod777/1 -> Mux/777
  "IW{2,1}(778,:)'"/1 -> dotprod778/1
  dotprod778/1 -> Mux/778
  "IW{2,1}(779,:)'"/1 -> dotprod779/1
  dotprod779/1 -> Mux/779
  "IW{2,1}(780,:)'"/1 -> dotprod780/1
  dotprod780/1 -> Mux/780
  "IW{2,1}(781,:)'"/1 -> dotprod781/1
  dotprod781/1 -> Mux/781
  "IW{2,1}(782,:)'"/1 -> dotprod782/1
  dotprod782/1 -> Mux/782
  "IW{2,1}(783,:)'"/1 -> dotprod783/1
  dotprod783/1 -> Mux/783
  "IW{2,1}(784,:)'"/1 -> dotprod784/1
  dotprod784/1 -> Mux/784
  "IW{2,1}(785,:)'"/1 -> dotprod785/1
  dotprod785/1 -> Mux/785
  "IW{2,1}(786,:)'"/1 -> dotprod786/1
  dotprod786/1 -> Mux/786
  "IW{2,1}(787,:)'"/1 -> dotprod787/1
  dotprod787/1 -> Mux/787
  "IW{2,1}(788,:)'"/1 -> dotprod788/1
  dotprod788/1 -> Mux/788
  "IW{2,1}(789,:)'"/1 -> dotprod789/1
  dotprod789/1 -> Mux/789
  "IW{2,1}(790,:)'"/1 -> dotprod790/1
  dotprod790/1 -> Mux/790
  "IW{2,1}(791,:)'"/1 -> dotprod791/1
  dotprod791/1 -> Mux/791
  "IW{2,1}(792,:)'"/1 -> dotprod792/1
  dotprod792/1 -> Mux/792
  "IW{2,1}(793,:)'"/1 -> dotprod793/1
  dotprod793/1 -> Mux/793
  "IW{2,1}(794,:)'"/1 -> dotprod794/1
  dotprod794/1 -> Mux/794
  "IW{2,1}(795,:)'"/1 -> dotprod795/1
  dotprod795/1 -> Mux/795
  "IW{2,1}(796,:)'"/1 -> dotprod796/1
  dotprod796/1 -> Mux/796
  "IW{2,1}(797,:)'"/1 -> dotprod797/1
  dotprod797/1 -> Mux/797
  "IW{2,1}(798,:)'"/1 -> dotprod798/1
  dotprod798/1 -> Mux/798
  "IW{2,1}(799,:)'"/1 -> dotprod799/1
  dotprod799/1 -> Mux/799
  "IW{2,1}(800,:)'"/1 -> dotprod800/1
  dotprod800/1 -> Mux/800
  "IW{2,1}(801,:)'"/1 -> dotprod801/1
  dotprod801/1 -> Mux/801
  "IW{2,1}(802,:)'"/1 -> dotprod802/1
  dotprod802/1 -> Mux/802
  "IW{2,1}(803,:)'"/1 -> dotprod803/1
  dotprod803/1 -> Mux/803
  "IW{2,1}(804,:)'"/1 -> dotprod804/1
  dotprod804/1 -> Mux/804
  "IW{2,1}(805,:)'"/1 -> dotprod805/1
  dotprod805/1 -> Mux/805
  "IW{2,1}(806,:)'"/1 -> dotprod806/1
  dotprod806/1 -> Mux/806
  "IW{2,1}(807,:)'"/1 -> dotprod807/1
  dotprod807/1 -> Mux/807
  "IW{2,1}(808,:)'"/1 -> dotprod808/1
  dotprod808/1 -> Mux/808
  "IW{2,1}(809,:)'"/1 -> dotprod809/1
  dotprod809/1 -> Mux/809
  "IW{2,1}(810,:)'"/1 -> dotprod810/1
  dotprod810/1 -> Mux/810
  "IW{2,1}(811,:)'"/1 -> dotprod811/1
  dotprod811/1 -> Mux/811
  "IW{2,1}(812,:)'"/1 -> dotprod812/1
  dotprod812/1 -> Mux/812
  "IW{2,1}(813,:)'"/1 -> dotprod813/1
  dotprod813/1 -> Mux/813
  "IW{2,1}(814,:)'"/1 -> dotprod814/1
  dotprod814/1 -> Mux/814
  "IW{2,1}(815,:)'"/1 -> dotprod815/1
  dotprod815/1 -> Mux/815
  "IW{2,1}(816,:)'"/1 -> dotprod816/1
  dotprod816/1 -> Mux/816
  "IW{2,1}(817,:)'"/1 -> dotprod817/1
  dotprod817/1 -> Mux/817
  "IW{2,1}(818,:)'"/1 -> dotprod818/1
  dotprod818/1 -> Mux/818
  "IW{2,1}(819,:)'"/1 -> dotprod819/1
  dotprod819/1 -> Mux/819
  "IW{2,1}(820,:)'"/1 -> dotprod820/1
  dotprod820/1 -> Mux/820
  "IW{2,1}(821,:)'"/1 -> dotprod821/1
  dotprod821/1 -> Mux/821
  "IW{2,1}(822,:)'"/1 -> dotprod822/1
  dotprod822/1 -> Mux/822
  "IW{2,1}(823,:)'"/1 -> dotprod823/1
  dotprod823/1 -> Mux/823
  "IW{2,1}(824,:)'"/1 -> dotprod824/1
  dotprod824/1 -> Mux/824
  "IW{2,1}(825,:)'"/1 -> dotprod825/1
  dotprod825/1 -> Mux/825
  "IW{2,1}(826,:)'"/1 -> dotprod826/1
  dotprod826/1 -> Mux/826
  "IW{2,1}(827,:)'"/1 -> dotprod827/1
  dotprod827/1 -> Mux/827
  "IW{2,1}(828,:)'"/1 -> dotprod828/1
  dotprod828/1 -> Mux/828
  "IW{2,1}(829,:)'"/1 -> dotprod829/1
  dotprod829/1 -> Mux/829
  "IW{2,1}(830,:)'"/1 -> dotprod830/1
  dotprod830/1 -> Mux/830
  "IW{2,1}(831,:)'"/1 -> dotprod831/1
  dotprod831/1 -> Mux/831
  "IW{2,1}(832,:)'"/1 -> dotprod832/1
  dotprod832/1 -> Mux/832
  "IW{2,1}(833,:)'"/1 -> dotprod833/1
  dotprod833/1 -> Mux/833
  "IW{2,1}(834,:)'"/1 -> dotprod834/1
  dotprod834/1 -> Mux/834
  "IW{2,1}(835,:)'"/1 -> dotprod835/1
  dotprod835/1 -> Mux/835
  "IW{2,1}(836,:)'"/1 -> dotprod836/1
  dotprod836/1 -> Mux/836
  "IW{2,1}(837,:)'"/1 -> dotprod837/1
  dotprod837/1 -> Mux/837
  "IW{2,1}(838,:)'"/1 -> dotprod838/1
  dotprod838/1 -> Mux/838
  "IW{2,1}(839,:)'"/1 -> dotprod839/1
  dotprod839/1 -> Mux/839
  "IW{2,1}(840,:)'"/1 -> dotprod840/1
  dotprod840/1 -> Mux/840
  "IW{2,1}(841,:)'"/1 -> dotprod841/1
  dotprod841/1 -> Mux/841
  "IW{2,1}(842,:)'"/1 -> dotprod842/1
  dotprod842/1 -> Mux/842
  "IW{2,1}(843,:)'"/1 -> dotprod843/1
  dotprod843/1 -> Mux/843
  "IW{2,1}(844,:)'"/1 -> dotprod844/1
  dotprod844/1 -> Mux/844
  "IW{2,1}(845,:)'"/1 -> dotprod845/1
  dotprod845/1 -> Mux/845
  "IW{2,1}(846,:)'"/1 -> dotprod846/1
  dotprod846/1 -> Mux/846
  "IW{2,1}(847,:)'"/1 -> dotprod847/1
  dotprod847/1 -> Mux/847
  "IW{2,1}(848,:)'"/1 -> dotprod848/1
  dotprod848/1 -> Mux/848
  "IW{2,1}(849,:)'"/1 -> dotprod849/1
  dotprod849/1 -> Mux/849
  "IW{2,1}(850,:)'"/1 -> dotprod850/1
  dotprod850/1 -> Mux/850
  "IW{2,1}(851,:)'"/1 -> dotprod851/1
  dotprod851/1 -> Mux/851
  "IW{2,1}(852,:)'"/1 -> dotprod852/1
  dotprod852/1 -> Mux/852
  "IW{2,1}(853,:)'"/1 -> dotprod853/1
  dotprod853/1 -> Mux/853
  "IW{2,1}(854,:)'"/1 -> dotprod854/1
  dotprod854/1 -> Mux/854
  "IW{2,1}(855,:)'"/1 -> dotprod855/1
  dotprod855/1 -> Mux/855
  "IW{2,1}(856,:)'"/1 -> dotprod856/1
  dotprod856/1 -> Mux/856
  "IW{2,1}(857,:)'"/1 -> dotprod857/1
  dotprod857/1 -> Mux/857
  "IW{2,1}(858,:)'"/1 -> dotprod858/1
  dotprod858/1 -> Mux/858
  "IW{2,1}(859,:)'"/1 -> dotprod859/1
  dotprod859/1 -> Mux/859
  "IW{2,1}(860,:)'"/1 -> dotprod860/1
  dotprod860/1 -> Mux/860
  "IW{2,1}(861,:)'"/1 -> dotprod861/1
  dotprod861/1 -> Mux/861
  "IW{2,1}(862,:)'"/1 -> dotprod862/1
  dotprod862/1 -> Mux/862
  "IW{2,1}(863,:)'"/1 -> dotprod863/1
  dotprod863/1 -> Mux/863
  "IW{2,1}(864,:)'"/1 -> dotprod864/1
  dotprod864/1 -> Mux/864
  "IW{2,1}(865,:)'"/1 -> dotprod865/1
  dotprod865/1 -> Mux/865
  "IW{2,1}(866,:)'"/1 -> dotprod866/1
  dotprod866/1 -> Mux/866
  "IW{2,1}(867,:)'"/1 -> dotprod867/1
  dotprod867/1 -> Mux/867
  "IW{2,1}(868,:)'"/1 -> dotprod868/1
  dotprod868/1 -> Mux/868
  "IW{2,1}(869,:)'"/1 -> dotprod869/1
  dotprod869/1 -> Mux/869
  "IW{2,1}(870,:)'"/1 -> dotprod870/1
  dotprod870/1 -> Mux/870
  "IW{2,1}(871,:)'"/1 -> dotprod871/1
  dotprod871/1 -> Mux/871
  "IW{2,1}(872,:)'"/1 -> dotprod872/1
  dotprod872/1 -> Mux/872
  "IW{2,1}(873,:)'"/1 -> dotprod873/1
  dotprod873/1 -> Mux/873
  "IW{2,1}(874,:)'"/1 -> dotprod874/1
  dotprod874/1 -> Mux/874
  "IW{2,1}(875,:)'"/1 -> dotprod875/1
  dotprod875/1 -> Mux/875
  "IW{2,1}(876,:)'"/1 -> dotprod876/1
  dotprod876/1 -> Mux/876
  "IW{2,1}(877,:)'"/1 -> dotprod877/1
  dotprod877/1 -> Mux/877
  "IW{2,1}(878,:)'"/1 -> dotprod878/1
  dotprod878/1 -> Mux/878
  "IW{2,1}(879,:)'"/1 -> dotprod879/1
  dotprod879/1 -> Mux/879
  "IW{2,1}(880,:)'"/1 -> dotprod880/1
  dotprod880/1 -> Mux/880
  "IW{2,1}(881,:)'"/1 -> dotprod881/1
  dotprod881/1 -> Mux/881
  "IW{2,1}(882,:)'"/1 -> dotprod882/1
  dotprod882/1 -> Mux/882
  "IW{2,1}(883,:)'"/1 -> dotprod883/1
  dotprod883/1 -> Mux/883
  "IW{2,1}(884,:)'"/1 -> dotprod884/1
  dotprod884/1 -> Mux/884
  "IW{2,1}(885,:)'"/1 -> dotprod885/1
  dotprod885/1 -> Mux/885
  "IW{2,1}(886,:)'"/1 -> dotprod886/1
  dotprod886/1 -> Mux/886
  "IW{2,1}(887,:)'"/1 -> dotprod887/1
  dotprod887/1 -> Mux/887
  "IW{2,1}(888,:)'"/1 -> dotprod888/1
  dotprod888/1 -> Mux/888
  "IW{2,1}(889,:)'"/1 -> dotprod889/1
  dotprod889/1 -> Mux/889
  "IW{2,1}(890,:)'"/1 -> dotprod890/1
  dotprod890/1 -> Mux/890
  "IW{2,1}(891,:)'"/1 -> dotprod891/1
  dotprod891/1 -> Mux/891
  "IW{2,1}(892,:)'"/1 -> dotprod892/1
  dotprod892/1 -> Mux/892
  "IW{2,1}(893,:)'"/1 -> dotprod893/1
  dotprod893/1 -> Mux/893
  "IW{2,1}(894,:)'"/1 -> dotprod894/1
  dotprod894/1 -> Mux/894
  "IW{2,1}(895,:)'"/1 -> dotprod895/1
  dotprod895/1 -> Mux/895
  "IW{2,1}(896,:)'"/1 -> dotprod896/1
  dotprod896/1 -> Mux/896
  "IW{2,1}(897,:)'"/1 -> dotprod897/1
  dotprod897/1 -> Mux/897
  "IW{2,1}(898,:)'"/1 -> dotprod898/1
  dotprod898/1 -> Mux/898
  "IW{2,1}(899,:)'"/1 -> dotprod899/1
  dotprod899/1 -> Mux/899
  "IW{2,1}(900,:)'"/1 -> dotprod900/1
  dotprod900/1 -> Mux/900
  "IW{2,1}(901,:)'"/1 -> dotprod901/1
  dotprod901/1 -> Mux/901
  "IW{2,1}(902,:)'"/1 -> dotprod902/1
  dotprod902/1 -> Mux/902
  "IW{2,1}(903,:)'"/1 -> dotprod903/1
  dotprod903/1 -> Mux/903
  "IW{2,1}(904,:)'"/1 -> dotprod904/1
  dotprod904/1 -> Mux/904
  "IW{2,1}(905,:)'"/1 -> dotprod905/1
  dotprod905/1 -> Mux/905
  "IW{2,1}(906,:)'"/1 -> dotprod906/1
  dotprod906/1 -> Mux/906
  "IW{2,1}(907,:)'"/1 -> dotprod907/1
  dotprod907/1 -> Mux/907
  "IW{2,1}(908,:)'"/1 -> dotprod908/1
  dotprod908/1 -> Mux/908
  "IW{2,1}(909,:)'"/1 -> dotprod909/1
  dotprod909/1 -> Mux/909
  "IW{2,1}(910,:)'"/1 -> dotprod910/1
  dotprod910/1 -> Mux/910
  "IW{2,1}(911,:)'"/1 -> dotprod911/1
  dotprod911/1 -> Mux/911
  "IW{2,1}(912,:)'"/1 -> dotprod912/1
  dotprod912/1 -> Mux/912
  "IW{2,1}(913,:)'"/1 -> dotprod913/1
  dotprod913/1 -> Mux/913
  "IW{2,1}(914,:)'"/1 -> dotprod914/1
  dotprod914/1 -> Mux/914
  "IW{2,1}(915,:)'"/1 -> dotprod915/1
  dotprod915/1 -> Mux/915
  "IW{2,1}(916,:)'"/1 -> dotprod916/1
  dotprod916/1 -> Mux/916
  "IW{2,1}(917,:)'"/1 -> dotprod917/1
  dotprod917/1 -> Mux/917
  "IW{2,1}(918,:)'"/1 -> dotprod918/1
  dotprod918/1 -> Mux/918
  "IW{2,1}(919,:)'"/1 -> dotprod919/1
  dotprod919/1 -> Mux/919
  "IW{2,1}(920,:)'"/1 -> dotprod920/1
  dotprod920/1 -> Mux/920
  "IW{2,1}(921,:)'"/1 -> dotprod921/1
  dotprod921/1 -> Mux/921
  "IW{2,1}(922,:)'"/1 -> dotprod922/1
  dotprod922/1 -> Mux/922
  "IW{2,1}(923,:)'"/1 -> dotprod923/1
  dotprod923/1 -> Mux/923
  "IW{2,1}(924,:)'"/1 -> dotprod924/1
  dotprod924/1 -> Mux/924
  "IW{2,1}(925,:)'"/1 -> dotprod925/1
  dotprod925/1 -> Mux/925
  "IW{2,1}(926,:)'"/1 -> dotprod926/1
  dotprod926/1 -> Mux/926
  "IW{2,1}(927,:)'"/1 -> dotprod927/1
  dotprod927/1 -> Mux/927
  "IW{2,1}(928,:)'"/1 -> dotprod928/1
  dotprod928/1 -> Mux/928
  "IW{2,1}(929,:)'"/1 -> dotprod929/1
  dotprod929/1 -> Mux/929
  "IW{2,1}(930,:)'"/1 -> dotprod930/1
  dotprod930/1 -> Mux/930
  "IW{2,1}(931,:)'"/1 -> dotprod931/1
  dotprod931/1 -> Mux/931
  "IW{2,1}(932,:)'"/1 -> dotprod932/1
  dotprod932/1 -> Mux/932
  "IW{2,1}(933,:)'"/1 -> dotprod933/1
  dotprod933/1 -> Mux/933
  "IW{2,1}(934,:)'"/1 -> dotprod934/1
  dotprod934/1 -> Mux/934
  "IW{2,1}(935,:)'"/1 -> dotprod935/1
  dotprod935/1 -> Mux/935
  "IW{2,1}(936,:)'"/1 -> dotprod936/1
  dotprod936/1 -> Mux/936
  "IW{2,1}(937,:)'"/1 -> dotprod937/1
  dotprod937/1 -> Mux/937
  "IW{2,1}(938,:)'"/1 -> dotprod938/1
  dotprod938/1 -> Mux/938
  "IW{2,1}(939,:)'"/1 -> dotprod939/1
  dotprod939/1 -> Mux/939
  "IW{2,1}(940,:)'"/1 -> dotprod940/1
  dotprod940/1 -> Mux/940
  "IW{2,1}(941,:)'"/1 -> dotprod941/1
  dotprod941/1 -> Mux/941
  "IW{2,1}(942,:)'"/1 -> dotprod942/1
  dotprod942/1 -> Mux/942
  "IW{2,1}(943,:)'"/1 -> dotprod943/1
  dotprod943/1 -> Mux/943
  "IW{2,1}(944,:)'"/1 -> dotprod944/1
  dotprod944/1 -> Mux/944
  "IW{2,1}(945,:)'"/1 -> dotprod945/1
  dotprod945/1 -> Mux/945
  "IW{2,1}(946,:)'"/1 -> dotprod946/1
  dotprod946/1 -> Mux/946
  "IW{2,1}(947,:)'"/1 -> dotprod947/1
  dotprod947/1 -> Mux/947
  "IW{2,1}(948,:)'"/1 -> dotprod948/1
  dotprod948/1 -> Mux/948
  "IW{2,1}(949,:)'"/1 -> dotprod949/1
  dotprod949/1 -> Mux/949
  "IW{2,1}(950,:)'"/1 -> dotprod950/1
  dotprod950/1 -> Mux/950
  "IW{2,1}(951,:)'"/1 -> dotprod951/1
  dotprod951/1 -> Mux/951
  "IW{2,1}(952,:)'"/1 -> dotprod952/1
  dotprod952/1 -> Mux/952
  "IW{2,1}(953,:)'"/1 -> dotprod953/1
  dotprod953/1 -> Mux/953
  "IW{2,1}(954,:)'"/1 -> dotprod954/1
  dotprod954/1 -> Mux/954
  "IW{2,1}(955,:)'"/1 -> dotprod955/1
  dotprod955/1 -> Mux/955
  "IW{2,1}(956,:)'"/1 -> dotprod956/1
  dotprod956/1 -> Mux/956
  "IW{2,1}(957,:)'"/1 -> dotprod957/1
  dotprod957/1 -> Mux/957
  "IW{2,1}(958,:)'"/1 -> dotprod958/1
  dotprod958/1 -> Mux/958
  "IW{2,1}(959,:)'"/1 -> dotprod959/1
  dotprod959/1 -> Mux/959
  "IW{2,1}(960,:)'"/1 -> dotprod960/1
  dotprod960/1 -> Mux/960
  "IW{2,1}(961,:)'"/1 -> dotprod961/1
  dotprod961/1 -> Mux/961
  "IW{2,1}(962,:)'"/1 -> dotprod962/1
  dotprod962/1 -> Mux/962
  "IW{2,1}(963,:)'"/1 -> dotprod963/1
  dotprod963/1 -> Mux/963
  "IW{2,1}(964,:)'"/1 -> dotprod964/1
  dotprod964/1 -> Mux/964
  "IW{2,1}(965,:)'"/1 -> dotprod965/1
  dotprod965/1 -> Mux/965
  "IW{2,1}(966,:)'"/1 -> dotprod966/1
  dotprod966/1 -> Mux/966
  "IW{2,1}(967,:)'"/1 -> dotprod967/1
  dotprod967/1 -> Mux/967
  "IW{2,1}(968,:)'"/1 -> dotprod968/1
  dotprod968/1 -> Mux/968
  "IW{2,1}(969,:)'"/1 -> dotprod969/1
  dotprod969/1 -> Mux/969
  "IW{2,1}(970,:)'"/1 -> dotprod970/1
  dotprod970/1 -> Mux/970
  "IW{2,1}(971,:)'"/1 -> dotprod971/1
  dotprod971/1 -> Mux/971
  "IW{2,1}(972,:)'"/1 -> dotprod972/1
  dotprod972/1 -> Mux/972
  "IW{2,1}(973,:)'"/1 -> dotprod973/1
  dotprod973/1 -> Mux/973
  "IW{2,1}(974,:)'"/1 -> dotprod974/1
  dotprod974/1 -> Mux/974
  "IW{2,1}(975,:)'"/1 -> dotprod975/1
  dotprod975/1 -> Mux/975
  "IW{2,1}(976,:)'"/1 -> dotprod976/1
  dotprod976/1 -> Mux/976
  "IW{2,1}(977,:)'"/1 -> dotprod977/1
  dotprod977/1 -> Mux/977
  "IW{2,1}(978,:)'"/1 -> dotprod978/1
  dotprod978/1 -> Mux/978
  "IW{2,1}(979,:)'"/1 -> dotprod979/1
  dotprod979/1 -> Mux/979
  "IW{2,1}(980,:)'"/1 -> dotprod980/1
  dotprod980/1 -> Mux/980
  "IW{2,1}(981,:)'"/1 -> dotprod981/1
  dotprod981/1 -> Mux/981
  "IW{2,1}(982,:)'"/1 -> dotprod982/1
  dotprod982/1 -> Mux/982
  "IW{2,1}(983,:)'"/1 -> dotprod983/1
  dotprod983/1 -> Mux/983
  "IW{2,1}(984,:)'"/1 -> dotprod984/1
  dotprod984/1 -> Mux/984
  "IW{2,1}(985,:)'"/1 -> dotprod985/1
  dotprod985/1 -> Mux/985
  "IW{2,1}(986,:)'"/1 -> dotprod986/1
  dotprod986/1 -> Mux/986
  "IW{2,1}(987,:)'"/1 -> dotprod987/1
  dotprod987/1 -> Mux/987
  "IW{2,1}(988,:)'"/1 -> dotprod988/1
  dotprod988/1 -> Mux/988
  "IW{2,1}(989,:)'"/1 -> dotprod989/1
  dotprod989/1 -> Mux/989
  "IW{2,1}(990,:)'"/1 -> dotprod990/1
  dotprod990/1 -> Mux/990
  "IW{2,1}(991,:)'"/1 -> dotprod991/1
  dotprod991/1 -> Mux/991
  "IW{2,1}(992,:)'"/1 -> dotprod992/1
  dotprod992/1 -> Mux/992
  "IW{2,1}(993,:)'"/1 -> dotprod993/1
  dotprod993/1 -> Mux/993
  "IW{2,1}(994,:)'"/1 -> dotprod994/1
  dotprod994/1 -> Mux/994
  "IW{2,1}(995,:)'"/1 -> dotprod995/1
  dotprod995/1 -> Mux/995
  "IW{2,1}(996,:)'"/1 -> dotprod996/1
  dotprod996/1 -> Mux/996
  "IW{2,1}(997,:)'"/1 -> dotprod997/1
  dotprod997/1 -> Mux/997
  "IW{2,1}(998,:)'"/1 -> dotprod998/1
  dotprod998/1 -> Mux/998
  "IW{2,1}(999,:)'"/1 -> dotprod999/1
  dotprod999/1 -> Mux/999
  "IW{2,1}(1000,:)'"/1 -> dotprod1000/1
  dotprod1000/1 -> Mux/1000
  "IW{2,1}(1001,:)'"/1 -> dotprod1001/1
  dotprod1001/1 -> Mux/1001
  Mux/1 -> "lz{2,1}"/1
